simulink model "ScaraRobotApresentacao2023"  (R2024a)
settings: Solver=VariableStepAuto  StartTime=0.0  StopTime=200  RelTol=1e-3
model workspace: external: MATLAB File C:\Users\lucas\OneDrive\Documents\MATLAB\Robotica_2023b\ScaraRobot_DataFile.m (data not in the file)
values from neighbouring files (symbols this model uses):
  I = cell(1,n)    [calcularDinamica.m]    (also in inicializacaoAntropomorfico.m = {I1, I2, I3, I4, I5, I6, I7})
  L = [L1, L2, L3, L4, L5, L6, L7]    [inicializacaoAntropomorfico.m]
  Lcm = {Lcm1, Lcm2, Lcm3, Lcm4, Lcm5, Lcm6, Lcm7}    [inicializacaoAntropomorfico.m]
  m = [m1, m2, m3, m4, m5, m6, m7]    [inicializacaoAntropomorfico.m]
  Pf = [  0.05    [inicializacaoAntropomorfico.m]
  Pi = [  0.2    [inicializacaoAntropomorfico.m]
  Raio = [0]    [inicializacaoAntropomorfico.m]
  Sentido = [0]    [inicializacaoAntropomorfico.m]
  Tipo = [1]    [inicializacaoAntropomorfico.m]
undefined symbols (not defined in the file or in its folder): Lx1, Lx2, smiData, X, Y, Z
libraries: sm_lib x25, nesl_utility x5
(part 2 of 10)

== matlab function ScaraRobotApresentacao2023/Dinamica/MATLAB Function ==
  data: M output; I parameter; L parameter; Lcm parameter; Q input
function M = func_M(I, L, Lcm, Q)
%func_M
%    OUT1 = func_M(Ixx2,Ixx3,Ixx4,Ixx5,Ixx6,Ixy2,Ixy3,Ixy4,Ixy5,Ixy6,Ixz2,Ixz3,Ixz4,Ixz5,Ixz6,Iyx2,Iyx3,Iyx4,Iyx5,Iyx6,Iyy2,Iyy3,Iyy4,Iyy5,Iyy6,Iyz2,Iyz3,Iyz4,Iyz5,Iyz6,Izx2,Izx3,Izx4,Izx5,Izx6,Izy2,Izy3,Izy4,Izy5,Izy6,Izz1,Izz2,Izz3,Izz4,Izz5,Izz6,Lx2,Lx3,Lxcm1,Lxcm2,Lxcm3,Lxcm4,Lxcm5,Lxcm6,Lycm1,Lycm2,Lycm3,Lycm4,Lycm5,Lycm6,Lz4,Lz5,Lzcm2,Lzcm3,Lzcm4,Lzcm5,Lzcm6,Q1,Q2,Q3,Q4,Q5,Q6,M1,M2,M3,M4,M5,M6)
    
%    This function was generated by the Symbolic Math Toolbox version 24.1.
%    30-Apr-2025 07:30:44

Q1  = Q(1);
Q2  = Q(2);
Q3  = Q(3);
Q4  = Q(4);
Q5  = Q(5);
Q6  = Q(6);

Lx1 = L{1}(1);
Ly1 = L{1}(2);
Lz1 = L{1}(3);

Lx2 = L{2}(1);
Ly2 = L{2}(2);
Lz2 = L{2}(3);

Lx3 = L{3}(1);
Ly3 = L{3}(2);
Lz3 = L{3}(3);

Lx4 = L{4}(1);
Ly4 = L{4}(2);
Lz4 = L{4}(3);

Lx5 = L{5}(1);
Ly5 = L{5}(2);
Lz5 = L{5}(3);

Lx6 = L{6}(1);
Ly6 = L{6}(2);
Lz6 = L{6}(3);

Lxcm1 = Lcm{1}(1);
Lycm1 = Lcm{1}(2);
Lzcm1 = Lcm{1}(3);

Lxcm2 = Lcm{2}(1);
Lycm2 = Lcm{2}(2);
Lzcm2 = Lcm{2}(3);

Lxcm3 = Lcm{3}(1);
Lycm3 = Lcm{3}(2);
Lzcm3 = Lcm{3}(3);

Lxcm4 = Lcm{4}(1);
Lycm4 = Lcm{4}(2);
Lzcm4 = Lcm{4}(3);

Lxcm5 = Lcm{5}(1);
Lycm5 = Lcm{5}(2);
Lzcm5 = Lcm{5}(3);

Lxcm6 = Lcm{6}(1);
Lycm6 = Lcm{6}(2);
Lzcm6 = Lcm{6}(3);

Ixx1 = I{1}(1,1);
Ixy1 = I{1}(1,2);
Ixz1 = I{1}(1,3);
Iyx1 = I{1}(2,1);
Iyy1 = I{1}(2,2);
Iyz1 = I{1}(2,3);
Izx1 = I{1}(3,1);
Izy1 = I{1}(3,2);
Izz1 = I{1}(3,3);

Ixx2 = I{2}(1,1);
Ixy2 = I{2}(1,2);
Ixz2 = I{2}(1,3);
Iyx2 = I{2}(2,1);
Iyy2 = I{2}(2,2);
Iyz2 = I{2}(2,3);
Izx2 = I{2}(3,1);
Izy2 = I{2}(3,2);
Izz2 = I{2}(3,3);

Ixx3 = I{3}(1,1);
Ixy3 = I{3}(1,2);
Ixz3 = I{3}(1,3);
Iyx3 = I{3}(2,1);
Iyy3 = I{3}(2,2);
Iyz3 = I{3}(2,3);
Izx3 = I{3}(3,1);
Izy3 = I{3}(3,2);
Izz3 = I{3}(3,3);

Ixx4 = I{4}(1,1);
Ixy4 = I{4}(1,2);
Ixz4 = I{4}(1,3);
Iyx4 = I{4}(2,1);
Iyy4 = I{4}(2,2);
Iyz4 = I{4}(2,3);
Izx4 = I{4}(3,1);
Izy4 = I{4}(3,2);
Izz4 = I{4}(3,3);

Ixx5 = I{5}(1,1);
Ixy5 = I{5}(1,2);
Ixz5 = I{5}(1,3);
Iyx5 = I{5}(2,1);
Iyy5 = I{5}(2,2);
Iyz5 = I{5}(2,3);
Izx5 = I{5}(3,1);
Izy5 = I{5}(3,2);
Izz5 = I{5}(3,3);

Ixx6 = I{6}(1,1);
Ixy6 = I{6}(1,2);
Ixz6 = I{6}(1,3);
Iyx6 = I{6}(2,1);
Iyy6 = I{6}(2,2);
Iyz6 = I{6}(2,3);
Izx6 = I{6}(3,1);
Izy6 = I{6}(3,2);
Izz6 = I{6}(3,3);


t2 = cos(Q1);
t3 = cos(Q2);
t4 = cos(Q3);
t5 = cos(Q4);
t6 = cos(Q5);
t7 = cos(Q6);
t8 = sin(Q1);
t9 = sin(Q2);
t10 = sin(Q3);
t11 = sin(Q4);
t12 = sin(Q5);
t13 = sin(Q6);
t14 = Q2+Q3;
t15 = Lx2.^2;
t16 = Lx3.^2;
t17 = Lxcm3.^2;
t18 = Lxcm4.^2;
t19 = Lxcm5.^2;
t20 = Lxcm6.^2;
t21 = Lycm4.^2;
t22 = Lycm5.^2;
t23 = Lycm6.^2;
t24 = Lz4.^2;
t25 = Lz5.^2;
t26 = Lzcm3.^2;
t27 = Lzcm4.^2;
t28 = Lzcm5.^2;
t29 = Lzcm6.^2;
t30 = Q4.*2.0;
t31 = Q5.*2.0;
t32 = Q6.*2.0;
t45 = Lz5.*Lzcm6.*m6.*2.0;
t33 = cos(t32);
t34 = t5.^2;
t35 = t6.^2;
t36 = t7.^2;
t37 = sin(t30);
t38 = sin(t31);
t39 = sin(t32);
t40 = Ixx6.*t5;
t41 = Iyy5.*t5;
t42 = Izz6.*t6;
t43 = cos(t14);
t44 = sin(t14);
t46 = m4.*t16;
t47 = m5.*t16;
t48 = m6.*t16;
t49 = m3.*t17;
t50 = m5.*t19;
t51 = m6.*t20;
t52 = m4.*t21;
t53 = m5.*t22;
t54 = m6.*t23;
t55 = m5.*t24;
t56 = m6.*t24;
t57 = m6.*t25;
t58 = m3.*t26;
t59 = m4.*t27;
t60 = m5.*t28;
t61 = m6.*t29;
t62 = t2.*t5;
t63 = t2.*t11;
t64 = t5.*t8;
t65 = t8.*t11;
t66 = Ixx5.*t3.*t4;
t67 = Iyy6.*t3.*t4;
t68 = Izz4.*t3.*t4;
t69 = Lx2.*t2.*t3;
t70 = Lx2.*Lx3.*m4.*t4;
t71 = Lx2.*Lx3.*m5.*t4;
t72 = Lx2.*Lx3.*m6.*t4;
t73 = Lx2.*Lxcm3.*m3.*t4;
t74 = Lx3.*Lxcm5.*m5.*t6;
t75 = Lycm5.*Lz4.*m5.*t5;
t76 = Lycm6.*Lz5.*m6.*t7;
t77 = Lycm2.*Lzcm2.*m2.*t3;
t78 = Lycm4.*Lzcm4.*m4.*t5;
t79 = Lycm5.*Lzcm5.*m5.*t6;
t80 = Lycm6.*Lzcm6.*m6.*t7;
t81 = Lx2.*t3.*t8;
t82 = Lx2.*Lycm3.*m3.*t9;
t83 = Lxcm2.*Lycm2.*m2.*t9;
t84 = Lxcm5.*Lycm5.*m5.*t12;
t85 = Lxcm6.*Lycm6.*m6.*t12;
t86 = Lx2.*Lz4.*m5.*t10;
t87 = Lx2.*Lz4.*m6.*t10;
t88 = Lx3.*Lz5.*m6.*t12;
t89 = Lx2.*Lzcm3.*m3.*t10;
t90 = Lx2.*Lzcm4.*m4.*t10;
t91 = Lx3.*Lzcm5.*m5.*t12;
t92 = Lx3.*Lzcm6.*m6.*t12;
t93 = Lxcm6.*Lz5.*m6.*t13;
t94 = Lxcm4.*Lzcm4.*m4.*t11;
t95 = Lxcm5.*Lzcm5.*m5.*t11;
t96 = Lxcm6.*Lzcm6.*m6.*t13;
t97 = Ixx5.*t9.*t10;
t98 = Iyy6.*t9.*t10;
t99 = Izz4.*t9.*t10;
t100 = Izz6.*t11.*t12;
t111 = Lx3.*Lxcm4.*m4.*t5.*2.0;
t112 = Lz4.*Lz5.*m6.*t6.*2.0;
t113 = Lz4.*Lzcm5.*m5.*t6.*2.0;
t114 = Lz4.*Lzcm6.*m6.*t6.*2.0;
t115 = t5.*t45;
t116 = Lx3.*Lycm4.*m4.*t11.*2.0;
t117 = Lx3.*Lycm5.*m5.*t11.*2.0;
t118 = Lxcm5.*Lz4.*m5.*t12.*2.0;
t126 = (Iyz2.*t3)./2.0;
t127 = (Iyz4.*t5)./2.0;
t128 = (Iyz5.*t6)./2.0;
t129 = (Iyz6.*t7)./2.0;
t130 = (Izy2.*t3)./2.0;
t131 = (Izy4.*t5)./2.0;
t132 = (Izy5.*t6)./2.0;
t133 = (Izy6.*t7)./2.0;
t134 = (Ixy2.*t9)./2.0;
t135 = (Ixy5.*t12)./2.0;
t136 = (Ixy6.*t12)./2.0;
t137 = (Ixz4.*t11)./2.0;
t138 = (Ixz5.*t11)./2.0;
t139 = (Ixz6.*t13)./2.0;
t140 = (Iyx2.*t9)./2.0;
t141 = (Iyx5.*t12)./2.0;
t142 = (Iyx6.*t12)./2.0;
t143 = (Izx4.*t11)./2.0;
t144 = (Izx5.*t11)./2.0;
t145 = (Izx6.*t13)./2.0;
t147 = t2.*t3.*t4;
t149 = t2.*t3.*t10;
t150 = t2.*t4.*t9;
t151 = t3.*t4.*t8;
t152 = t2.*t9.*t10;
t153 = t3.*t8.*t10;
t154 = t4.*t8.*t9;
t155 = t8.*t9.*t10;
t203 = Lx2.*Lxcm4.*m4.*t3.*t5;
t204 = Lx2.*Lxcm4.*m4.*t4.*t5;
t205 = Lx2.*Lxcm5.*m5.*t4.*t6;
t206 = Lx3.*Lxcm6.*m6.*t6.*t7;
t207 = Lycm6.*Lz4.*m6.*t5.*t7;
t210 = Lycm3.*Lzcm3.*m3.*t3.*t4;
t214 = Lz4.*Lz5.*m6.*t5.*t6;
t215 = Lz4.*Lzcm5.*m5.*t5.*t6;
t216 = Lz4.*Lzcm6.*m6.*t5.*t6;
t217 = Ixy5.*t5.*t6.*t11;
t218 = Ixy6.*t5.*t6.*t11;
t219 = Ixy6.*t5.*t7.*t13;
t220 = Ixz6.*t6.*t7.*t12;
t221 = Iyx5.*t5.*t6.*t11;
t222 = Iyx6.*t5.*t6.*t11;
t223 = Iyx6.*t5.*t7.*t13;
t224 = Izx6.*t6.*t7.*t12;
t225 = Lx2.*Lycm4.*m4.*t3.*t11;
t226 = Lx2.*Lycm4.*m4.*t5.*t9;
t227 = Lx2.*Lycm4.*m4.*t4.*t11;
t228 = Lx2.*Lycm4.*m4.*t5.*t10;
t229 = Lx2.*Lycm5.*m5.*t3.*t11;
t230 = Lx2.*Lycm5.*m5.*t5.*t9;
t231 = Lx2.*Lycm5.*m5.*t4.*t11;
t232 = Lx2.*Lycm5.*m5.*t5.*t10;
t233 = Lx3.*Lycm6.*m6.*t6.*t13;
t234 = Lx3.*Lycm6.*m6.*t7.*t12;
t235 = Lxcm3.*Lycm3.*m3.*t3.*t10;
t236 = Lxcm3.*Lycm3.*m3.*t4.*t9;
t237 = Lxcm4.*Lycm4.*m4.*t3.*t10;
t238 = Lxcm4.*Lycm4.*m4.*t4.*t9;
t240 = Lxcm5.*Lycm5.*m5.*t6.*t11;
t242 = Lxcm6.*Lycm6.*m6.*t6.*t11;
t243 = Lx2.*Lz5.*m6.*t4.*t12;
t244 = Lx2.*Lz5.*m6.*t6.*t10;
t245 = Lx2.*Lzcm5.*m5.*t4.*t12;
t246 = Lx2.*Lzcm5.*m5.*t6.*t10;
t247 = Lx2.*Lzcm6.*m6.*t4.*t12;
t248 = Lx2.*Lzcm6.*m6.*t6.*t10;
t249 = Lxcm5.*Lz4.*m5.*t5.*t12;
t250 = Lxcm5.*Lz4.*m5.*t6.*t11;
t251 = Lxcm6.*Lz4.*m6.*t5.*t13;
t252 = Lxcm6.*Lz4.*m6.*t7.*t11;
t254 = Lxcm6.*Lz5.*m6.*t7.*t11;
t256 = Lxcm6.*Lz5.*m6.*t7.*t12;
t258 = Lxcm6.*Lzcm6.*m6.*t7.*t11;
t260 = Lxcm6.*Lzcm6.*m6.*t7.*t12;
t261 = Ixx6.*t3.*t10.*t11;
t262 = Ixx6.*t4.*t9.*t11;
t263 = Ixx5.*t6.*t11.*t12;
t264 = Ixx6.*t7.*t12.*t13;
t265 = Iyy5.*t3.*t10.*t11;
t266 = Iyy5.*t4.*t9.*t11;
t267 = Iyy6.*t6.*t11.*t12;
t268 = Iyy6.*t7.*t12.*t13;
t269 = Iyz5.*t5.*t11.*t12;
t270 = Iyz6.*t6.*t12.*t13;
t271 = Izy5.*t5.*t11.*t12;
t272 = Izy6.*t6.*t12.*t13;
t274 = Izz5.*t6.*t11.*t12;
t276 = Lx2.*Lxcm4.*m4.*t9.*t11;
t277 = Lx2.*Lxcm4.*m4.*t10.*t11;
t278 = Lx2.*Lxcm5.*m5.*t10.*t12;
t279 = Lx3.*Lxcm6.*m6.*t12.*t13;
t280 = Lycm6.*Lz4.*m6.*t11.*t13;
t281 = Lycm6.*Lz5.*m6.*t11.*t13;
t282 = Lycm6.*Lz5.*m6.*t12.*t13;
t283 = Lycm3.*Lzcm3.*m3.*t9.*t10;
t284 = Lycm5.*Lzcm5.*m5.*t11.*t12;
t285 = Lycm6.*Lzcm6.*m6.*t11.*t13;
t286 = Lycm6.*Lzcm6.*m6.*t12.*t13;
t287 = Lz4.*Lz5.*m6.*t11.*t12;
t288 = Lz4.*Lzcm5.*m5.*t11.*t12;
t289 = Lz4.*Lzcm6.*m6.*t11.*t12;
t290 = m4.*t9.*t10.*t18;
t299 = (Iyz3.*t3.*t4)./2.0;
t303 = (Izy3.*t3.*t4)./2.0;
t307 = (Ixy3.*t3.*t10)./2.0;
t308 = (Ixy3.*t4.*t9)./2.0;
t309 = (Ixy4.*t3.*t10)./2.0;
t310 = (Ixy4.*t4.*t9)./2.0;
t312 = (Ixy5.*t6.*t11)./2.0;
t314 = (Ixy6.*t6.*t11)./2.0;
t316 = (Ixz6.*t7.*t11)./2.0;
t318 = (Ixz6.*t7.*t12)./2.0;
t319 = (Iyx3.*t3.*t10)./2.0;
t320 = (Iyx3.*t4.*t9)./2.0;
t321 = (Iyx4.*t3.*t10)./2.0;
t322 = (Iyx4.*t4.*t9)./2.0;
t324 = (Iyx5.*t6.*t11)./2.0;
t326 = (Iyx6.*t6.*t11)./2.0;
t328 = (Izx6.*t7.*t11)./2.0;
t330 = (Izx6.*t7.*t12)./2.0;
t331 = (Iyz3.*t9.*t10)./2.0;
t332 = (Iyz5.*t11.*t12)./2.0;
t333 = (Iyz6.*t11.*t13)./2.0;
t334 = (Iyz6.*t12.*t13)./2.0;
t335 = (Izy3.*t9.*t10)./2.0;
t336 = (Izy5.*t11.*t12)./2.0;
t337 = (Izy6.*t11.*t13)./2.0;
t338 = (Izy6.*t12.*t13)./2.0;
t366 = t3.*t4.*t45;
t367 = Lx3.*Lycm6.*m6.*t7.*t11.*2.0;
t371 = Lxcm6.*Lz4.*m6.*t7.*t12.*2.0;
t372 = m4.*t3.*t4.*t18;
t379 = Lx3.*Lxcm6.*m6.*t11.*t13.*2.0;
t380 = Lycm6.*Lz4.*m6.*t12.*t13.*2.0;
t381 = t9.*t10.*t45;
t383 = Iyz5.*t5.*t6.*(-1.0./2.0);
t384 = Iyz6.*t5.*t7.*(-1.0./2.0);
t385 = Iyz6.*t6.*t7.*(-1.0./2.0);
t387 = Izy5.*t5.*t6.*(-1.0./2.0);
t388 = Izy6.*t5.*t7.*(-1.0./2.0);
t389 = Izy6.*t6.*t7.*(-1.0./2.0);
t393 = Ixy6.*t5.*t12.*(-1.0./2.0);
t394 = Ixz6.*t5.*t13.*(-1.0./2.0);
t395 = Ixz6.*t6.*t13.*(-1.0./2.0);
t399 = Iyx6.*t5.*t12.*(-1.0./2.0);
t400 = Izx6.*t5.*t13.*(-1.0./2.0);
t401 = Izx6.*t6.*t13.*(-1.0./2.0);
t441 = Lx3.*Lxcm4.*m4.*t3.*t4.*t5;
t442 = Lx2.*Lxcm5.*m5.*t3.*t5.*t6;
t444 = Lx2.*Lxcm6.*m6.*t3.*t5.*t7;
t445 = Lx2.*Lxcm6.*m6.*t4.*t6.*t7;
t454 = Ixy6.*t3.*t4.*t7.*t13;
t455 = Ixz5.*t3.*t4.*t6.*t12;
t456 = Iyx6.*t3.*t4.*t7.*t13;
t457 = Izx5.*t3.*t4.*t6.*t12;
t458 = Lx3.*Lycm4.*m4.*t3.*t4.*t11;
t459 = Lx3.*Lycm4.*m4.*t3.*t5.*t10;
t460 = Lx3.*Lycm4.*m4.*t4.*t5.*t9;
t461 = Lx3.*Lycm5.*m5.*t3.*t4.*t11;
t462 = Lx3.*Lycm5.*m5.*t3.*t5.*t10;
t463 = Lx3.*Lycm5.*m5.*t4.*t5.*t9;
t464 = Lx2.*Lycm6.*m6.*t3.*t5.*t13;
t465 = Lx2.*Lycm6.*m6.*t3.*t7.*t11;
t466 = Lx2.*Lycm6.*m6.*t5.*t7.*t9;
t467 = Lx2.*Lycm6.*m6.*t4.*t7.*t11;
t468 = Lx2.*Lycm6.*m6.*t5.*t7.*t10;
t469 = Lx2.*Lycm6.*m6.*t4.*t6.*t13;
t470 = Lx2.*Lycm6.*m6.*t4.*t7.*t12;
t472 = Lxcm5.*Lycm5.*m5.*t3.*t6.*t10;
t473 = Lxcm5.*Lycm5.*m5.*t4.*t6.*t9;
t475 = Lxcm6.*Lycm6.*m6.*t3.*t6.*t10;
t476 = Lxcm6.*Lycm6.*m6.*t4.*t6.*t9;
t477 = Lx2.*Lz5.*m6.*t3.*t5.*t12;
t478 = Lx2.*Lz5.*m6.*t3.*t6.*t11;
t481 = Lx2.*Lzcm5.*m5.*t3.*t5.*t12;
t482 = Lx2.*Lzcm5.*m5.*t3.*t6.*t11;
t485 = Lx2.*Lzcm6.*m6.*t3.*t5.*t12;
t486 = Lx2.*Lzcm6.*m6.*t3.*t6.*t11;
t490 = Lxcm6.*Lz4.*m6.*t5.*t7.*t12;
t495 = Lxcm4.*Lzcm4.*m4.*t3.*t5.*t10;
t496 = Lxcm4.*Lzcm4.*m4.*t4.*t5.*t9;
t498 = Lxcm5.*Lzcm5.*m5.*t3.*t5.*t10;
t499 = Lxcm5.*Lzcm5.*m5.*t4.*t5.*t9;
t502 = Ixx4.*t3.*t5.*t10.*t11;
t503 = Ixx4.*t4.*t5.*t9.*t11;
t507 = Ixx6.*t6.*t7.*t11.*t13;
t508 = Iyy4.*t3.*t5.*t10.*t11;
t509 = Iyy4.*t4.*t5.*t9.*t11;
t513 = Iyy6.*t6.*t7.*t11.*t13;
t514 = Iyz6.*t5.*t7.*t11.*t12;
t515 = Izy6.*t5.*t7.*t11.*t12;
t516 = Izz5.*t3.*t5.*t10.*t11;
t517 = Izz5.*t4.*t5.*t9.*t11;
t518 = Izz6.*t3.*t5.*t10.*t11;
t519 = Izz6.*t4.*t5.*t9.*t11;
t520 = Izz6.*t3.*t5.*t10.*t12;
t521 = Izz6.*t4.*t5.*t9.*t12;
t522 = Lx3.*Lxcm4.*m4.*t3.*t10.*t11;
t523 = Lx3.*Lxcm4.*m4.*t4.*t9.*t11;
t524 = Lx3.*Lxcm4.*m4.*t5.*t9.*t10;
t525 = Lx2.*Lxcm5.*m5.*t3.*t11.*t12;
t526 = Lx2.*Lxcm5.*m5.*t6.*t9.*t11;
t528 = Lx2.*Lxcm5.*m5.*t6.*t10.*t11;
t529 = Lx2.*Lxcm6.*m6.*t3.*t11.*t13;
t530 = Lx2.*Lxcm6.*m6.*t5.*t9.*t13;
t531 = Lx2.*Lxcm6.*m6.*t4.*t11.*t13;
t532 = Lx2.*Lxcm6.*m6.*t5.*t10.*t13;
t533 = Lx2.*Lxcm6.*m6.*t7.*t10.*t11;
t534 = Lx2.*Lxcm6.*m6.*t4.*t12.*t13;
t535 = Lx2.*Lxcm6.*m6.*t7.*t10.*t12;
t536 = Lycm5.*Lz4.*m5.*t3.*t10.*t11;
t537 = Lycm5.*Lz4.*m5.*t4.*t9.*t11;
t539 = Lycm6.*Lz4.*m6.*t5.*t12.*t13;
t543 = Lycm4.*Lzcm4.*m4.*t3.*t10.*t11;
t544 = Lycm4.*Lzcm4.*m4.*t4.*t9.*t11;
t546 = Lycm5.*Lzcm5.*m5.*t3.*t10.*t12;
t547 = Lycm5.*Lzcm5.*m5.*t4.*t9.*t12;
t551 = Ixy6.*t7.*t9.*t10.*t13;
t552 = Ixz5.*t6.*t9.*t10.*t12;
t553 = Ixz6.*t5.*t11.*t12.*t13;
t554 = Iyx6.*t7.*t9.*t10.*t13;
t555 = Izx5.*t6.*t9.*t10.*t12;
t556 = Izx6.*t5.*t11.*t12.*t13;
t557 = Lx3.*Lycm4.*m4.*t9.*t10.*t11;
t558 = Lx3.*Lycm5.*m5.*t9.*t10.*t11;
t559 = Lx2.*Lycm6.*m6.*t10.*t11.*t13;
t560 = Lx2.*Lycm6.*m6.*t10.*t12.*t13;
t563 = Lx2.*Lz5.*m6.*t9.*t11.*t12;
t564 = Lx2.*Lz5.*m6.*t10.*t11.*t12;
t565 = Lx2.*Lzcm5.*m5.*t9.*t11.*t12;
t566 = Lx2.*Lzcm5.*m5.*t10.*t11.*t12;
t567 = Lx2.*Lzcm6.*m6.*t9.*t11.*t12;
t568 = Lx2.*Lzcm6.*m6.*t10.*t11.*t12;
t637 = Lz5.*Lzcm6.*m6.*t9.*t10.*-2.0;
t661 = Lxcm6.*Lycm6.*m6.*t5.*t7.*t13.*2.0;
t669 = t3.*t10.*t11.*t45;
t670 = t4.*t9.*t11.*t45;
t698 = (Ixy5.*t3.*t6.*t10)./2.0;
t699 = (Ixy5.*t4.*t6.*t9)./2.0;
t701 = (Ixy6.*t3.*t6.*t10)./2.0;
t702 = (Ixy6.*t4.*t6.*t9)./2.0;
t704 = (Ixz4.*t3.*t5.*t10)./2.0;
t705 = (Ixz4.*t4.*t5.*t9)./2.0;
t707 = (Ixz5.*t3.*t5.*t10)./2.0;
t708 = (Ixz5.*t4.*t5.*t9)./2.0;
t712 = (Iyx5.*t3.*t6.*t10)./2.0;
t713 = (Iyx5.*t4.*t6.*t9)./2.0;
t715 = (Iyx6.*t3.*t6.*t10)./2.0;
t716 = (Iyx6.*t4.*t6.*t9)./2.0;
t718 = (Izx4.*t3.*t5.*t10)./2.0;
t719 = (Izx4.*t4.*t5.*t9)./2.0;
t721 = (Izx5.*t3.*t5.*t10)./2.0;
t722 = (Izx5.*t4.*t5.*t9)./2.0;
t725 = (Iyz4.*t3.*t10.*t11)./2.0;
t726 = (Iyz4.*t4.*t9.*t11)./2.0;
t728 = (Iyz5.*t3.*t10.*t12)./2.0;
t729 = (Iyz5.*t4.*t9.*t12)./2.0;
t733 = (Izy4.*t3.*t10.*t11)./2.0;
t734 = (Izy4.*t4.*t9.*t11)./2.0;
t736 = (Izy5.*t3.*t10.*t12)./2.0;
t737 = (Izy5.*t4.*t9.*t12)./2.0;
t765 = Lx3.*Lxcm6.*m6.*t3.*t4.*t5.*t7;
t778 = Lx3.*Lycm6.*m6.*t3.*t4.*t5.*t13;
t779 = Lx3.*Lycm6.*m6.*t3.*t4.*t7.*t11;
t780 = Lx3.*Lycm6.*m6.*t3.*t5.*t7.*t10;
t781 = Lx3.*Lycm6.*m6.*t4.*t5.*t7.*t9;
t793 = Lx3.*Lz5.*m6.*t3.*t4.*t6.*t11;
t795 = Lx3.*Lzcm5.*m5.*t3.*t4.*t6.*t11;
t797 = Lxcm5.*Lz4.*m5.*t3.*t5.*t6.*t10;
t798 = Lxcm5.*Lz4.*m5.*t4.*t5.*t6.*t9;
t800 = Lx3.*Lzcm6.*m6.*t3.*t4.*t6.*t11;
t802 = Lxcm6.*Lz4.*m6.*t3.*t5.*t7.*t10;
t803 = Lxcm6.*Lz4.*m6.*t4.*t5.*t7.*t9;
t805 = Lxcm6.*Lz5.*m6.*t3.*t5.*t7.*t10;
t806 = Lxcm6.*Lz5.*m6.*t4.*t5.*t7.*t9;
t810 = Lxcm6.*Lzcm6.*m6.*t3.*t5.*t7.*t10;
t811 = Lxcm6.*Lzcm6.*m6.*t4.*t5.*t7.*t9;
t815 = Ixx5.*t3.*t5.*t6.*t10.*t12;
t816 = Ixx5.*t4.*t5.*t6.*t9.*t12;
t818 = Ixx6.*t3.*t6.*t7.*t10.*t13;
t819 = Ixx6.*t4.*t6.*t7.*t9.*t13;
t821 = Iyy6.*t3.*t5.*t6.*t10.*t12;
t822 = Iyy6.*t4.*t5.*t6.*t9.*t12;
t824 = Iyy6.*t3.*t6.*t7.*t10.*t13;
t825 = Iyy6.*t4.*t6.*t7.*t9.*t13;
t829 = Izz5.*t3.*t5.*t6.*t10.*t12;
t830 = Izz5.*t4.*t5.*t6.*t9.*t12;
t834 = Lx3.*Lxcm5.*m5.*t3.*t4.*t11.*t12;
t838 = Lx3.*Lxcm6.*m6.*t3.*t4.*t11.*t13;
t839 = Lx3.*Lxcm6.*m6.*t3.*t5.*t10.*t13;
t840 = Lx3.*Lxcm6.*m6.*t4.*t5.*t9.*t13;
t841 = Lx3.*Lxcm6.*m6.*t5.*t7.*t9.*t10;
t843 = Lx2.*Lxcm6.*m6.*t3.*t7.*t11.*t12;
t844 = Lx2.*Lxcm6.*m6.*t6.*t7.*t9.*t11;
t848 = Lycm6.*Lz4.*m6.*t3.*t5.*t10.*t13;
t849 = Lycm6.*Lz4.*m6.*t3.*t7.*t10.*t11;
t850 = Lycm6.*Lz4.*m6.*t4.*t5.*t9.*t13;
t851 = Lycm6.*Lz4.*m6.*t4.*t7.*t9.*t11;
t854 = Lycm6.*Lz5.*m6.*t3.*t5.*t10.*t13;
t856 = Lycm6.*Lz5.*m6.*t4.*t5.*t9.*t13;
t868 = Lycm6.*Lzcm6.*m6.*t3.*t5.*t10.*t13;
t870 = Lycm6.*Lzcm6.*m6.*t4.*t5.*t9.*t13;
t877 = Lz4.*Lz5.*m6.*t3.*t5.*t10.*t12;
t878 = Lz4.*Lz5.*m6.*t3.*t6.*t10.*t11;
t879 = Lz4.*Lz5.*m6.*t4.*t5.*t9.*t12;
t880 = Lz4.*Lz5.*m6.*t4.*t6.*t9.*t11;
t882 = Lz4.*Lzcm5.*m5.*t3.*t5.*t10.*t12;
t883 = Lz4.*Lzcm5.*m5.*t3.*t6.*t10.*t11;
t884 = Lz4.*Lzcm5.*m5.*t4.*t5.*t9.*t12;
t885 = Lz4.*Lzcm5.*m5.*t4.*t6.*t9.*t11;
t887 = Lz4.*Lzcm6.*m6.*t3.*t5.*t10.*t12;
t888 = Lz4.*Lzcm6.*m6.*t3.*t6.*t10.*t11;
t889 = Lz4.*Lzcm6.*m6.*t4.*t5.*t9.*t12;
t890 = Lz4.*Lzcm6.*m6.*t4.*t6.*t9.*t11;
t891 = Ixy6.*t3.*t7.*t10.*t11.*t13;
t892 = Ixy6.*t4.*t7.*t9.*t11.*t13;
t893 = Ixy6.*t6.*t7.*t11.*t12.*t13;
t895 = Iyx6.*t3.*t7.*t10.*t11.*t13;
t896 = Iyx6.*t4.*t7.*t9.*t11.*t13;
t897 = Iyx6.*t6.*t7.*t11.*t12.*t13;
t899 = Lx3.*Lycm6.*m6.*t5.*t9.*t10.*t13;
t900 = Lx3.*Lycm6.*m6.*t7.*t9.*t10.*t11;
t901 = Lx2.*Lycm6.*m6.*t3.*t11.*t12.*t13;
t902 = Lx2.*Lycm6.*m6.*t6.*t9.*t11.*t13;
t914 = Lx3.*Lz5.*m6.*t6.*t9.*t10.*t11;
t918 = Lx3.*Lzcm5.*m5.*t6.*t9.*t10.*t11;
t919 = Lxcm5.*Lz4.*m5.*t3.*t10.*t11.*t12;
t920 = Lxcm5.*Lz4.*m5.*t4.*t9.*t11.*t12;
t925 = Lx3.*Lzcm6.*m6.*t6.*t9.*t10.*t11;
t926 = Lxcm6.*Lz4.*m6.*t3.*t10.*t11.*t13;
t927 = Lxcm6.*Lz4.*m6.*t4.*t9.*t11.*t13;
t951 = Lx3.*Lxcm5.*m5.*t9.*t10.*t11.*t12;
t952 = Lx3.*Lxcm6.*m6.*t9.*t10.*t11.*t13;
t1023 = Lz5.*Lzcm6.*m6.*t6.*t11.*t12.*-2.0;
t1037 = Iyz4.*t3.*t4.*t5.*(-1.0./2.0);
t1038 = Iyz5.*t3.*t4.*t6.*(-1.0./2.0);
t1040 = Izy4.*t3.*t4.*t5.*(-1.0./2.0);
t1041 = Izy5.*t3.*t4.*t6.*(-1.0./2.0);
t1049 = Ixy6.*t3.*t4.*t12.*(-1.0./2.0);
t1050 = Ixz4.*t3.*t4.*t11.*(-1.0./2.0);
t1054 = Ixz6.*t6.*t7.*t11.*(-1.0./2.0);
t1057 = Iyx6.*t3.*t4.*t12.*(-1.0./2.0);
t1058 = Izx4.*t3.*t4.*t11.*(-1.0./2.0);
t1062 = Izx6.*t6.*t7.*t11.*(-1.0./2.0);
t1067 = Iyz6.*t7.*t11.*t12.*(-1.0./2.0);
t1072 = Izy6.*t7.*t11.*t12.*(-1.0./2.0);
t1095 = Ixy5.*t9.*t10.*t12.*(-1.0./2.0);
t1096 = Ixz5.*t9.*t10.*t11.*(-1.0./2.0);
t1097 = Ixz6.*t11.*t12.*t13.*(-1.0./2.0);
t1098 = Iyx5.*t9.*t10.*t12.*(-1.0./2.0);
t1099 = Izx5.*t9.*t10.*t11.*(-1.0./2.0);
t1100 = Izx6.*t11.*t12.*t13.*(-1.0./2.0);
t1124 = Lxcm6.*Lycm6.*m6.*t3.*t4.*t7.*t13.*2.0;
t1125 = Lxcm5.*Lzcm5.*m5.*t3.*t4.*t6.*t12.*2.0;
t1132 = Lxcm6.*Lycm6.*m6.*t7.*t9.*t10.*t13.*2.0;
t1134 = Lxcm5.*Lzcm5.*m5.*t6.*t9.*t10.*t12.*2.0;
t1136 = m4.*t3.*t5.*t10.*t11.*t18;
t1137 = m4.*t4.*t5.*t9.*t11.*t18;
t1169 = (Ixz6.*t3.*t5.*t7.*t10)./2.0;
t1170 = (Ixz6.*t4.*t5.*t7.*t9)./2.0;
t1180 = (Izx6.*t3.*t5.*t7.*t10)./2.0;
t1181 = (Izx6.*t4.*t5.*t7.*t9)./2.0;
t1191 = (Iyz6.*t3.*t5.*t10.*t13)./2.0;
t1193 = (Iyz6.*t4.*t5.*t9.*t13)./2.0;
t1205 = (Izy6.*t3.*t5.*t10.*t13)./2.0;
t1207 = (Izy6.*t4.*t5.*t9.*t13)./2.0;
t1286 = Lx3.*Lxcm6.*m6.*t3.*t4.*t7.*t11.*t12;
t1311 = Ixz5.*t3.*t5.*t6.*t10.*t11.*t12;
t1312 = Ixz5.*t4.*t5.*t6.*t9.*t11.*t12;
t1315 = Izx5.*t3.*t5.*t6.*t10.*t11.*t12;
t1316 = Izx5.*t4.*t5.*t6.*t9.*t11.*t12;
t1317 = Lx3.*Lycm6.*m6.*t3.*t4.*t11.*t12.*t13;
t1344 = Lx3.*Lxcm6.*m6.*t7.*t9.*t10.*t11.*t12;
t1354 = Lx3.*Lycm6.*m6.*t9.*t10.*t11.*t12.*t13;
t1466 = Ixy6.*t3.*t5.*t6.*t10.*(-1.0./2.0);
t1467 = Ixy6.*t4.*t5.*t6.*t9.*(-1.0./2.0);
t1472 = Iyx6.*t3.*t5.*t6.*t10.*(-1.0./2.0);
t1473 = Iyx6.*t4.*t5.*t6.*t9.*(-1.0./2.0);
t1478 = Iyz5.*t3.*t6.*t10.*t11.*(-1.0./2.0);
t1479 = Iyz5.*t4.*t6.*t9.*t11.*(-1.0./2.0);
t1480 = Iyz6.*t3.*t4.*t11.*t13.*(-1.0./2.0);
t1481 = Iyz6.*t3.*t7.*t10.*t11.*(-1.0./2.0);
t1482 = Iyz6.*t4.*t7.*t9.*t11.*(-1.0./2.0);
t1483 = Iyz6.*t3.*t4.*t12.*t13.*(-1.0./2.0);
t1484 = Iyz6.*t3.*t7.*t10.*t12.*(-1.0./2.0);
t1485 = Iyz6.*t4.*t7.*t9.*t12.*(-1.0./2.0);
t1486 = Izy5.*t3.*t6.*t10.*t11.*(-1.0./2.0);
t1487 = Izy5.*t4.*t6.*t9.*t11.*(-1.0./2.0);
t1488 = Izy6.*t3.*t4.*t11.*t13.*(-1.0./2.0);
t1489 = Izy6.*t3.*t7.*t10.*t11.*(-1.0./2.0);
t1490 = Izy6.*t4.*t7.*t9.*t11.*(-1.0./2.0);
t1491 = Izy6.*t3.*t4.*t12.*t13.*(-1.0./2.0);
M = ft_1({Ixx2,Ixx3,Ixx4,Ixx5,Ixx6,Ixy4,Ixy5,Ixy6,Ixz2,Ixz3,Ixz4,Ixz5,Ixz6,Iyx4,Iyx5,Iyx6,Iyy2,Iyy3,Iyy4,Iyy5,Iyy6,Iyz4,Iyz5,Iyz6,Izx2,Izx3,Izx4,Izx5,Izx6,Izy4,Izy5,Izy6,Izz1,Izz2,Izz3,Izz4,Izz5,Izz6,Lx3,Lxcm1,Lxcm2,Lxcm3,Lxcm4,Lxcm5,Lxcm6,Lycm1,Lycm2,Lycm3,Lycm4,Lycm5,Lycm6,Lz4,Lz5,Lzcm2,Lzcm3,Lzcm4,Lzcm5,Lzcm6,m1,m2,m3,m4,m5,m6,t10,t100,t1023,t1037,t1038,t1040,t1041,t1049,t1050,t1054,t1057,t1058,t1062,t1067,t1072,t1095,t1096,t1097,t1098,t1099,t11,t1100,t111,t112,t1124,t1125,t113,t1132,t1134,t1136,t1137,t114,t115,t116,t1169,t117,t1170,t118,t1180,t1181,t1191,t1193,t12,t1205,t1207,t126,t127,t128,t1286,t129,t13,t130,t131,t1311,t1312,t1315,t1316,t1317,t132,t133,t134,t1344,t135,t1354,t136,t137,t138,t139,t140,t141,t142,t143,t144,t145,t1466,t1467,t147,t1472,t1473,t1478,t1479,t1480,t1481,t1482,t1483,t1484,t1485,t1486,t1487,t1488,t1489,t149,t1490,t1491,t15,t150,t151,t152,t153,t154,t155,t18,t2,t203,t204,t205,t206,t207,t210,t214,t215,t216,t217,t218,t219,t220,t221,t222,t223,t224,t225,t226,t227,t228,t229,t230,t231,t232,t233,t234,t235,t236,t237,t238,t240,t242,t243,t244,t245,t246,t247,t248,t249,t250,t251,t252,t254,t256,t258,t260,t261,t262,t263,t264,t265,t266,t267,t268,t269,t270,t271,t272,t274,t276,t277,t278,t279,t280,t281,t282,t283,t284,t285,t286,t287,t288,t289,t290,t299,t3,t303,t307,t308,t309,t310,t312,t314,t316,t318,t319,t320,t321,t322,t324,t326,t328,t33,t330,t331,t332,t333,t334,t335,t336,t337,t338,t34,t35,t36,t366,t367,t37,t371,t372,t379,t38,t380,t381,t383,t384,t385,t387,t388,t389,t39,t393,t394,t395,t399,t4,t40,t400,t401,t41,t42,t43,t44,t441,t442,t444,t445,t45,t454,t455,t456,t457,t458,t459,t46,t460,t461,t462,t463,t464,t465,t466,t467,t468,t469,t47,t470,t472,t473,t475,t476,t477,t478,t48,t481,t482,t485,t486,t49,t490,t495,t496,t498,t499,t5,t50,t502,t503,t507,t508,t509,t51,t513,t514,t515,t516,t517,t518,t519,t52,t520,t521,t522,t523,t524,t525,t526,t528,t529,t53,t530,t531,t532,t533,t534,t535,t536,t537,t539,t54,t543,t544,t546,t547,t55,t551,t552,t553,t554,t555,t556,t557,t558,t559,t56,t560,t563,t564,t565,t566,t567,t568,t57,t58,t59,t6,t60,t61,t62,t63,t637,t64,t65,t66,t661,t669,t67,t670,t68,t69,t698,t699,t7,t70,t701,t702,t704,t705,t707,t708,t71,t712,t713,t715,t716,t718,t719,t72,t721,t722,t725,t726,t728,t729,t73,t733,t734,t736,t737,t74,t75,t76,t765,t77,t778,t779,t78,t780,t781,t79,t793,t795,t797,t798,t8,t80,t800,t802,t803,t805,t806,t81,t810,t811,t815,t816,t818,t819,t82,t821,t822,t824,t825,t829,t83,t830,t834,t838,t839,t84,t840,t841,t843,t844,t848,t849,t85,t850,t851,t854,t856,t86,t868,t87,t870,t877,t878,t879,t88,t880,t882,t883,t884,t885,t887,t888,t889,t89,t890,t891,t892,t893,t895,t896,t897,t899,t9,t90,t900,t901,t902,t91,t914,t918,t919,t92,t920,t925,t926,t927,t93,t94,t95,t951,t952,t96,t97,t98,t99});
end
function out1 = ft_1(ct)
[Ixx2,Ixx3,Ixx4,Ixx5,Ixx6,Ixy4,Ixy5,Ixy6,Ixz2,Ixz3,Ixz4,Ixz5,Ixz6,Iyx4,Iyx5,Iyx6,Iyy2,Iyy3,Iyy4,Iyy5,Iyy6,Iyz4,Iyz5,Iyz6,Izx2,Izx3,Izx4,Izx5,Izx6,Izy4,Izy5,Izy6,Izz1,Izz2,Izz3,Izz4,Izz5,Izz6,Lx3,Lxcm1,Lxcm2,Lxcm3,Lxcm4,Lxcm5,Lxcm6,Lycm1,Lycm2,Lycm3,Lycm4,Lycm5,Lycm6,Lz4,Lz5,Lzcm2,Lzcm3,Lzcm4,Lzcm5,Lzcm6,m1,m2,m3,m4,m5,m6,t10,t100,t1023,t1037,t1038,t1040,t1041,t1049,t1050,t1054,t1057,t1058,t1062,t1067,t1072,t1095,t1096,t1097,t1098,t1099,t11,t1100,t111,t112,t1124,t1125,t113,t1132,t1134,t1136,t1137,t114,t115,t116,t1169,t117,t1170,t118,t1180,t1181,t1191,t1193,t12,t1205,t1207,t126,t127,t128,t1286,t129,t13,t130,t131,t1311,t1312,t1315,t1316,t1317,t132,t133,t134,t1344,t135,t1354,t136,t137,t138,t139,t140,t141,t142,t143,t144,t145,t1466,t1467,t147,t1472,t1473,t1478,t1479,t1480,t1481,t1482,t1483,t1484,t1485,t1486,t1487,t1488,t1489,t149,t1490,t1491,t15,t150,t151,t152,t153,t154,t155,t18,t2,t203,t204,t205,t206,t207,t210,t214,t215,t216,t217,t218,t219,t220,t221,t222,t223,t224,t225,t226,t227,t228,t229,t230,t231,t232,t233,t234,t235,t236,t237,t238,t240,t242,t243,t244,t245,t246,t247,t248,t249,t250,t251,t252,t254,t256,t258,t260,t261,t262,t263,t264,t265,t266,t267,t268,t269,t270,t271,t272,t274,t276,t277,t278,t279,t280,t281,t282,t283,t284,t285,t286,t287,t288,t289,t290,t299,t3,t303,t307,t308,t309,t310,t312,t314,t316,t318,t319,t320,t321,t322,t324,t326,t328,t33,t330,t331,t332,t333,t334,t335,t336,t337,t338,t34,t35,t36,t366,t367,t37,t371,t372,t379,t38,t380,t381,t383,t384,t385,t387,t388,t389,t39,t393,t394,t395,t399,t4,t40,t400,t401,t41,t42,t43,t44,t441,t442,t444,t445,t45,t454,t455,t456,t457,t458,t459,t46,t460,t461,t462,t463,t464,t465,t466,t467,t468,t469,t47,t470,t472,t473,t475,t476,t477,t478,t48,t481,t482,t485,t486,t49,t490,t495,t496,t498,t499,t5,t50,t502,t503,t507,t508,t509,t51,t513,t514,t515,t516,t517,t518,t519,t52,t520,t521,t522,t523,t524,t525,t526,t528,t529,t53,t530,t531,t532,t533,t534,t535,t536,t537,t539,t54,t543,t544,t546,t547,t55,t551,t552,t553,t554,t555,t556,t557,t558,t559,t56,t560,t563,t564,t565,t566,t567,t568,t57,t58,t59,t6,t60,t61,t62,t63,t637,t64,t65,t66,t661,t669,t67,t670,t68,t69,t698,t699,t7,t70,t701,t702,t704,t705,t707,t708,t71,t712,t713,t715,t716,t718,t719,t72,t721,t722,t725,t726,t728,t729,t73,t733,t734,t736,t737,t74,t75,t76,t765,t77,t778,t779,t78,t780,t781,t79,t793,t795,t797,t798,t8,t80,t800,t802,t803,t805,t806,t81,t810,t811,t815,t816,t818,t819,t82,t821,t822,t824,t825,t829,t83,t830,t834,t838,t839,t84,t840,t841,t843,t844,t848,t849,t85,t850,t851,t854,t856,t86,t868,t87,t870,t877,t878,t879,t88,t880,t882,t883,t884,t885,t887,t888,t889,t89,t890,t891,t892,t893,t895,t896,t897,t899,t9,t90,t900,t901,t902,t91,t914,t918,t919,t92,t920,t925,t926,t927,t93,t94,t95,t951,t952,t96,t97,t98,t99] = ct{:};
t1492 = Izy6.*t3.*t7.*t10.*t12.*(-1.0./2.0);
t1493 = Izy6.*t4.*t7.*t9.*t12.*(-1.0./2.0);
t1509 = Ixy6.*t3.*t10.*t11.*t12.*(-1.0./2.0);
t1510 = Ixy6.*t4.*t9.*t11.*t12.*(-1.0./2.0);
t1511 = Ixz6.*t3.*t10.*t11.*t13.*(-1.0./2.0);
t1512 = Ixz6.*t4.*t9.*t11.*t13.*(-1.0./2.0);
t1513 = Ixz6.*t7.*t9.*t10.*t11.*(-1.0./2.0);
t1514 = Ixz6.*t3.*t10.*t12.*t13.*(-1.0./2.0);
t1515 = Ixz6.*t4.*t9.*t12.*t13.*(-1.0./2.0);
t1516 = Ixz6.*t7.*t9.*t10.*t12.*(-1.0./2.0);
t1518 = Iyx6.*t3.*t10.*t11.*t12.*(-1.0./2.0);
t1519 = Iyx6.*t4.*t9.*t11.*t12.*(-1.0./2.0);
t1520 = Izx6.*t3.*t10.*t11.*t13.*(-1.0./2.0);
t1521 = Izx6.*t4.*t9.*t11.*t13.*(-1.0./2.0);
t1522 = Izx6.*t7.*t9.*t10.*t11.*(-1.0./2.0);
t1523 = Izx6.*t3.*t10.*t12.*t13.*(-1.0./2.0);
t1524 = Izx6.*t4.*t9.*t12.*t13.*(-1.0./2.0);
t1525 = Izx6.*t7.*t9.*t10.*t12.*(-1.0./2.0);
t1610 = Lxcm6.*Lycm6.*m6.*t3.*t7.*t10.*t11.*t13.*2.0;
t1611 = Lxcm6.*Lycm6.*m6.*t4.*t7.*t9.*t11.*t13.*2.0;
t1782 = Iyz6.*t3.*t5.*t6.*t10.*t13.*(-1.0./2.0);
t1784 = Iyz6.*t4.*t5.*t6.*t9.*t13.*(-1.0./2.0);
t1786 = Izy6.*t3.*t5.*t6.*t10.*t13.*(-1.0./2.0);
t1788 = Izy6.*t4.*t5.*t6.*t9.*t13.*(-1.0./2.0);
t1986 = Lxcm6.*Lycm6.*m6.*t3.*t5.*t7.*t10.*t11.*t13.*-2.0;
t1987 = Lxcm6.*Lycm6.*m6.*t4.*t5.*t7.*t9.*t11.*t13.*-2.0;
t101 = Ixx4.*t34;
t102 = Ixx5.*t35;
t103 = Ixx6.*t34;
t104 = Iyy4.*t34;
t105 = Iyy5.*t34;
t106 = Iyy6.*t35;
t107 = Izz5.*t34;
t108 = Izz5.*t35;
t109 = Izz6.*t34;
t110 = Izz6.*t35;
t119 = t5.*t50;
t120 = t6.*t51;
t121 = t5.*t54;
t122 = t6.*t54;
t123 = t5.*t57;
t124 = t5.*t60;
t125 = t5.*t61;
t146 = t6.*t43;
t148 = t12.*t43;
t156 = -t62;
t157 = -t65;
t158 = -t75;
t159 = -t76;
t160 = -t77;
t161 = -t78;
t162 = -t79;
t163 = -t80;
t164 = -t116;
t165 = -t117;
t166 = -t85;
t167 = -t118;
t168 = -t93;
t169 = -t94;
t170 = -t96;
t171 = -t97;
t172 = -t98;
t173 = -t99;
t174 = -t126;
t175 = -t127;
t176 = -t128;
t177 = -t129;
t178 = -t130;
t179 = -t131;
t180 = -t132;
t181 = -t133;
t182 = -t136;
t183 = -t137;
t184 = -t139;
t185 = -t142;
t186 = -t143;
t187 = -t145;
t188 = t36.*t40;
t189 = Iyy6.*t5.*t36;
t190 = Ixy6.*t12.*t36;
t191 = Ixz5.*t11.*t35;
t192 = Iyx6.*t12.*t36;
t193 = Izx5.*t11.*t35;
t194 = Lxcm4.*Lycm4.*m4.*t37;
t195 = Lxcm6.*Lycm6.*m6.*t39;
t196 = Lxcm5.*Lzcm5.*m5.*t38;
t202 = t3.*t4.*t42;
t208 = t5.*t76;
t209 = t6.*t76;
t211 = t5.*t79;
t212 = t5.*t80;
t213 = t6.*t80;
t239 = t5.*t84;
t241 = t5.*t85;
t253 = t5.*t93;
t255 = t6.*t93;
t257 = t5.*t96;
t259 = t6.*t96;
t273 = t9.*t10.*t42;
t275 = t11.*t12.*t42;
t291 = t9.*t10.*t51;
t292 = t11.*t12.*t51;
t293 = t9.*t10.*t52;
t294 = t9.*t10.*t53;
t295 = t11.*t12.*t54;
t296 = t9.*t10.*t57;
t297 = t9.*t10.*t60;
t298 = t9.*t10.*t61;
t300 = t5.*t128;
t301 = t5.*t129;
t302 = t6.*t129;
t304 = t5.*t132;
t305 = t5.*t133;
t306 = t6.*t133;
t311 = t5.*t135;
t313 = t5.*t136;
t315 = t5.*t139;
t317 = t6.*t139;
t323 = t5.*t141;
t325 = t5.*t142;
t327 = t5.*t145;
t329 = t6.*t145;
t339 = t5.*t6.*t44;
t340 = t5.*t12.*t44;
t341 = t7.*t11.*t44;
t342 = t11.*t13.*t44;
t343 = t34.*t45;
t344 = t35.*t45;
t345 = m4.*t18.*t34;
t346 = t35.*t50;
t347 = t34.*t51;
t348 = t34.*t52;
t349 = t34.*t53;
t350 = t35.*t54;
t351 = t34.*t57;
t352 = t35.*t57;
t353 = t34.*t60;
t354 = t35.*t60;
t355 = t34.*t61;
t356 = t35.*t61;
t357 = -t152;
t358 = -t155;
t359 = (Ixy4.*t37)./2.0;
t360 = (Ixy6.*t39)./2.0;
t361 = (Ixz5.*t38)./2.0;
t362 = (Iyx4.*t37)./2.0;
t363 = (Iyx6.*t39)./2.0;
t364 = (Izx5.*t38)./2.0;
t365 = t5.*t74.*2.0;
t368 = t5.*t88.*2.0;
t369 = t5.*t91.*2.0;
t370 = t5.*t92.*2.0;
t373 = t3.*t4.*t51;
t374 = t3.*t4.*t52;
t375 = t3.*t4.*t53;
t376 = t3.*t4.*t57;
t377 = t3.*t4.*t60;
t378 = t3.*t4.*t61;
t382 = -t299;
t386 = -t303;
t390 = -t309;
t391 = -t310;
t392 = -t312;
t396 = -t321;
t397 = -t322;
t398 = -t324;
t402 = t35.*t66;
t403 = Ixx6.*t3.*t4.*t36;
t404 = t35.*t67;
t405 = t36.*t67;
t408 = -t332;
t409 = -t333;
t410 = -t334;
t411 = -t336;
t412 = -t337;
t413 = -t338;
t414 = Ixy4.*t3.*t10.*t34;
t415 = Ixy4.*t4.*t9.*t34;
t417 = Ixy6.*t6.*t11.*t36;
t418 = Ixy6.*t7.*t13.*t34;
t419 = Ixy6.*t7.*t13.*t35;
t420 = Ixz5.*t6.*t12.*t34;
t421 = Ixz6.*t7.*t11.*t35;
t422 = Iyx4.*t3.*t10.*t34;
t423 = Iyx4.*t4.*t9.*t34;
t425 = Iyx6.*t6.*t11.*t36;
t426 = Iyx6.*t7.*t13.*t34;
t427 = Iyx6.*t7.*t13.*t35;
t428 = Izx5.*t6.*t12.*t34;
t429 = Izx6.*t7.*t11.*t35;
t430 = t35.*t97;
t431 = Ixx6.*t9.*t10.*t36;
t432 = t35.*t98;
t433 = t36.*t98;
t434 = Iyz6.*t11.*t13.*t35;
t435 = Izy6.*t11.*t13.*t35;
t443 = t5.*t205;
t447 = t6.*t207;
t471 = t3.*t4.*t84;
t474 = t3.*t4.*t85;
t479 = t5.*t243;
t480 = t5.*t244;
t483 = t5.*t245;
t484 = t5.*t246;
t487 = t5.*t247;
t488 = t5.*t248;
t489 = t6.*t251;
t491 = t6.*t252;
t493 = t6.*t254;
t497 = t3.*t4.*t95;
t501 = t6.*t258;
t504 = t3.*t10.*t11.*t40;
t505 = t4.*t9.*t11.*t40;
t506 = t7.*t12.*t13.*t40;
t510 = t3.*t10.*t11.*t41;
t511 = t4.*t9.*t11.*t41;
t512 = t5.*t268;
t527 = t5.*t278;
t538 = t9.*t10.*t75;
t540 = t6.*t280;
t541 = t6.*t281;
t545 = t9.*t10.*t78;
t548 = t9.*t10.*t79;
t549 = t6.*t285;
t561 = t9.*t10.*t84;
t562 = t9.*t10.*t85;
t570 = t9.*t10.*t94;
t571 = t9.*t10.*t95;
t577 = -t207;
t580 = -t210;
t586 = Ixx6.*t35.*t36;
t588 = Iyy6.*t34.*t36;
t592 = -t217;
t593 = -t219;
t594 = -t220;
t595 = -t221;
t596 = -t223;
t597 = -t224;
t598 = -t225;
t599 = -t227;
t600 = -t228;
t601 = -t229;
t602 = -t231;
t603 = -t232;
t604 = -t233;
t605 = -t367;
t606 = -t234;
t607 = -t237;
t608 = -t238;
t609 = -t240;
t611 = -t249;
t612 = -t250;
t613 = -t251;
t614 = -t252;
t616 = -t371;
t620 = -t263;
t621 = -t264;
t622 = -t267;
t623 = -t269;
t624 = -t271;
t626 = -t277;
t627 = -t278;
t628 = -t379;
t629 = -t279;
t630 = -t281;
t631 = -t282;
t632 = -t284;
t633 = -t285;
t634 = -t286;
t635 = -t287;
t636 = -t288;
t638 = -t289;
t639 = -t290;
t646 = t36.*t85.*2.0;
t647 = t35.*t95.*2.0;
t648 = t5.*t36.*t51;
t652 = t5.*t206.*2.0;
t658 = t5.*t233.*2.0;
t659 = t5.*t240.*2.0;
t660 = t5.*t242.*2.0;
t662 = t6.*t256.*2.0;
t663 = t6.*t260.*2.0;
t666 = t6.*t282.*2.0;
t667 = t5.*t284.*2.0;
t668 = t6.*t286.*2.0;
t672 = t3.*t10.*t11.*t50;
t673 = t4.*t9.*t11.*t50;
t675 = t6.*t11.*t12.*t50;
t676 = t7.*t12.*t13.*t51;
t677 = t3.*t10.*t11.*t54;
t678 = t4.*t9.*t11.*t54;
t681 = t7.*t12.*t13.*t54;
t682 = t3.*t10.*t11.*t57;
t683 = t4.*t9.*t11.*t57;
t684 = t6.*t11.*t12.*t57;
t685 = t3.*t10.*t11.*t60;
t686 = t4.*t9.*t11.*t60;
t687 = t3.*t10.*t11.*t61;
t688 = t4.*t9.*t11.*t61;
t689 = t6.*t11.*t12.*t60;
t690 = t6.*t11.*t12.*t61;
t697 = t3.*t4.*t135;
t706 = t3.*t4.*t138;
t711 = t3.*t4.*t141;
t720 = t3.*t4.*t144;
t727 = t9.*t10.*t127;
t730 = t9.*t10.*t128;
t731 = t6.*t333;
t735 = t9.*t10.*t131;
t738 = t9.*t10.*t132;
t739 = t6.*t337;
t742 = t9.*t10.*t136;
t743 = t9.*t10.*t137;
t747 = t9.*t10.*t142;
t748 = t9.*t10.*t143;
t764 = t3.*t4.*t5.*t74;
t766 = t6.*t444;
t767 = t5.*t445;
t773 = t3.*t4.*t220;
t774 = t3.*t4.*t224;
t782 = t6.*t464;
t783 = t6.*t465;
t784 = t5.*t469;
t785 = t6.*t468;
t787 = t5.*t472;
t788 = t5.*t473;
t790 = t5.*t475;
t791 = t5.*t476;
t792 = t3.*t4.*t5.*t88;
t794 = t3.*t4.*t5.*t91;
t799 = t3.*t4.*t5.*t92;
t804 = t3.*t4.*t254;
t808 = t3.*t4.*t256;
t809 = t3.*t4.*t258;
t813 = t3.*t4.*t260;
t814 = t6.*t11.*t12.*t66;
t820 = t6.*t11.*t12.*t67;
t823 = t7.*t12.*t13.*t67;
t826 = t3.*t4.*t270;
t827 = t3.*t4.*t272;
t828 = t3.*t4.*t274;
t832 = t3.*t5.*t10.*t12.*t42;
t833 = t4.*t5.*t9.*t12.*t42;
t835 = t3.*t10.*t11.*t74;
t836 = t4.*t9.*t11.*t74;
t837 = t5.*t9.*t10.*t74;
t842 = t6.*t529;
t845 = t6.*t532;
t846 = t5.*t535;
t847 = t6.*t533;
t852 = t9.*t10.*t207;
t853 = t3.*t4.*t281;
t858 = t3.*t4.*t282;
t859 = t3.*t10.*t12.*t76;
t860 = t4.*t9.*t12.*t76;
t862 = t5.*t546;
t864 = t5.*t547;
t867 = t3.*t4.*t285;
t872 = t3.*t4.*t286;
t873 = t3.*t10.*t12.*t80;
t874 = t4.*t9.*t12.*t80;
t903 = t5.*t560;
t904 = t6.*t559;
t905 = t3.*t10.*t11.*t84;
t906 = t4.*t9.*t11.*t84;
t911 = t3.*t10.*t11.*t88;
t912 = t4.*t9.*t11.*t88;
t913 = t5.*t9.*t10.*t88;
t915 = t3.*t10.*t11.*t91;
t916 = t4.*t9.*t11.*t91;
t917 = t5.*t9.*t10.*t91;
t921 = t9.*t10.*t250;
t922 = t3.*t10.*t11.*t92;
t923 = t4.*t9.*t11.*t92;
t924 = t5.*t9.*t10.*t92;
t928 = t9.*t10.*t251;
t931 = t9.*t10.*t254;
t932 = t3.*t10.*t12.*t93;
t933 = t4.*t9.*t12.*t93;
t935 = t9.*t10.*t256;
t938 = t9.*t10.*t258;
t939 = t3.*t10.*t12.*t96;
t940 = t4.*t9.*t12.*t96;
t942 = t9.*t10.*t260;
t943 = t6.*t11.*t12.*t97;
t944 = t9.*t10.*t264;
t945 = t6.*t11.*t12.*t98;
t947 = t9.*t10.*t270;
t948 = t9.*t10.*t272;
t949 = t9.*t10.*t274;
t953 = t9.*t10.*t281;
t954 = t9.*t10.*t282;
t955 = t9.*t10.*t285;
t956 = t9.*t10.*t286;
t957 = t9.*t10.*t287;
t958 = t9.*t10.*t288;
t959 = t9.*t10.*t289;
t966 = -t458;
t967 = -t461;
t968 = -t464;
t969 = -t465;
t970 = -t467;
t971 = -t468;
t972 = -t469;
t973 = -t470;
t975 = -t472;
t976 = -t473;
t979 = -t661;
t981 = -t490;
t987 = -t498;
t988 = -t499;
t992 = -t502;
t993 = -t503;
t995 = -t513;
t996 = -t514;
t997 = -t515;
t998 = -t516;
t999 = -t517;
t1000 = -t518;
t1001 = -t519;
t1002 = -t520;
t1003 = -t521;
t1004 = -t524;
t1005 = -t525;
t1007 = -t528;
t1008 = -t529;
t1009 = -t531;
t1010 = -t532;
t1011 = -t533;
t1012 = -t534;
t1013 = -t535;
t1014 = -t536;
t1015 = -t537;
t1017 = -t543;
t1018 = -t544;
t1019 = -t546;
t1020 = -t547;
t1024 = -t551;
t1025 = -t552;
t1026 = -t553;
t1027 = -t554;
t1028 = -t555;
t1029 = -t556;
t1031 = -t564;
t1032 = -t566;
t1033 = -t568;
t1039 = t6.*t384;
t1042 = t6.*t388;
t1047 = -t698;
t1048 = -t699;
t1051 = -t707;
t1052 = -t708;
t1053 = t6.*t394;
t1055 = -t712;
t1056 = -t713;
t1059 = -t721;
t1060 = -t722;
t1061 = t6.*t400;
t1063 = -t725;
t1064 = -t726;
t1065 = -t728;
t1066 = -t729;
t1068 = -t733;
t1069 = -t734;
t1070 = -t736;
t1071 = -t737;
t1073 = Ixy5.*t3.*t6.*t10.*t34;
t1074 = Ixy5.*t4.*t6.*t9.*t34;
t1075 = Ixy6.*t3.*t6.*t10.*t34;
t1076 = Ixy6.*t4.*t6.*t9.*t34;
t1078 = Ixy6.*t3.*t6.*t10.*t36;
t1079 = Ixy6.*t4.*t6.*t9.*t36;
t1081 = Ixz5.*t3.*t5.*t10.*t35;
t1082 = Ixz5.*t4.*t5.*t9.*t35;
t1083 = t34.*t220;
t1084 = Iyx5.*t3.*t6.*t10.*t34;
t1085 = Iyx5.*t4.*t6.*t9.*t34;
t1086 = Iyx6.*t3.*t6.*t10.*t34;
t1087 = Iyx6.*t4.*t6.*t9.*t34;
t1089 = Iyx6.*t3.*t6.*t10.*t36;
t1090 = Iyx6.*t4.*t6.*t9.*t36;
t1092 = Izx5.*t3.*t5.*t10.*t35;
t1093 = Izx5.*t4.*t5.*t9.*t35;
t1094 = t34.*t224;
t1101 = t36.*t261;
t1102 = t36.*t262;
t1103 = Ixx6.*t6.*t11.*t12.*t36;
t1104 = Iyy6.*t3.*t10.*t11.*t36;
t1105 = Iyy6.*t4.*t9.*t11.*t36;
t1106 = t36.*t267;
t1107 = Iyz5.*t3.*t10.*t12.*t34;
t1108 = Iyz5.*t4.*t9.*t12.*t34;
t1109 = t34.*t270;
t1110 = Izy5.*t3.*t10.*t12.*t34;
t1111 = Izy5.*t4.*t9.*t12.*t34;
t1112 = t34.*t272;
t1113 = t35.*t281.*2.0;
t1114 = t35.*t285.*2.0;
t1119 = t9.*t10.*t36.*t54;
t1126 = t6.*t7.*t11.*t13.*t40.*2.0;
out1 = ft_2({Ixx2,Ixx3,Ixx4,Ixx5,Ixx6,Ixy4,Ixy5,Ixy6,Ixz2,Ixz3,Ixz4,Ixz5,Ixz6,Iyx4,Iyx5,Iyx6,Iyy2,Iyy3,Iyy4,Iyy5,Iyy6,Iyz4,Iyz5,Iyz6,Izx2,Izx3,Izx4,Izx5,Izx6,Izy4,Izy5,Izy6,Izz1,Izz2,Izz3,Izz4,Izz5,Izz6,Lx3,Lxcm1,Lxcm2,Lxcm3,Lxcm4,Lxcm5,Lxcm6,Lycm1,Lycm2,Lycm3,Lycm4,Lycm5,Lycm6,Lz4,Lz5,Lzcm2,Lzcm3,Lzcm4,Lzcm5,Lzcm6,m1,m2,m3,m4,m5,m6,t10,t100,t1000,t1001,t1002,t1003,t1004,t1005,t1007,t1008,t1009,t101,t1010,t1011,t1012,t1013,t1014,t1015,t1017,t1018,t1019,t102,t1020,t1023,t1024,t1025,t1026,t1027,t1028,t1029,t103,t1031,t1032,t1033,t1037,t1038,t1039,t104,t1040,t1041,t1042,t1047,t1048,t1049,t105,t1050,t1051,t1052,t1053,t1054,t1055,t1056,t1057,t1058,t1059,t106,t1060,t1061,t1062,t1063,t1064,t1065,t1066,t1067,t1068,t1069,t107,t1070,t1071,t1072,t1073,t1074,t1075,t1076,t1078,t1079,t108,t1081,t1082,t1083,t1084,t1085,t1086,t1087,t1089,t109,t1090,t1092,t1093,t1094,t1095,t1096,t1097,t1098,t1099,t11,t110,t1100,t1101,t1102,t1103,t1104,t1105,t1106,t1107,t1108,t1109,t111,t1110,t1111,t1112,t1113,t1114,t1119,t112,t1124,t1125,t1126,t113,t1132,t1134,t1136,t1137,t114,t115,t1169,t1170,t1180,t1181,t119,t1191,t1193,t12,t120,t1205,t1207,t121,t122,t123,t124,t125,t1286,t13,t1311,t1312,t1315,t1316,t1317,t134,t1344,t135,t1354,t138,t140,t141,t144,t146,t1466,t1467,t147,t1472,t1473,t1478,t1479,t148,t1480,t1481,t1482,t1483,t1484,t1485,t1486,t1487,t1488,t1489,t149,t1490,t1491,t1492,t1493,t15,t150,t1509,t151,t1510,t1511,t1512,t1513,t1514,t1515,t1516,t1518,t1519,t1520,t1521,t1522,t1523,t1524,t1525,t153,t154,t156,t157,t158,t159,t160,t161,t1610,t1611,t162,t163,t164,t165,t166,t167,t168,t169,t170,t171,t172,t173,t174,t175,t176,t177,t178,t1782,t1784,t1786,t1788,t179,t18,t180,t181,t182,t183,t184,t185,t186,t187,t188,t189,t190,t191,t192,t193,t194,t195,t196,t1986,t1987,t2,t202,t203,t204,t205,t206,t208,t209,t211,t212,t213,t214,t215,t216,t218,t219,t220,t222,t223,t224,t226,t227,t230,t231,t233,t235,t236,t237,t238,t239,t241,t242,t243,t244,t245,t246,t247,t248,t253,t254,t255,t256,t257,t258,t259,t260,t261,t262,t265,t266,t268,t270,t272,t273,t274,t275,t276,t278,t280,t282,t283,t286,t291,t292,t293,t294,t295,t296,t297,t298,t3,t300,t301,t302,t304,t305,t306,t307,t308,t311,t313,t314,t315,t316,t317,t318,t319,t320,t323,t325,t326,t327,t328,t329,t33,t330,t331,t333,t334,t335,t337,t338,t339,t34,t340,t341,t342,t343,t344,t345,t346,t347,t348,t349,t35,t350,t351,t352,t353,t354,t355,t356,t357,t358,t359,t36,t360,t361,t362,t363,t364,t365,t366,t368,t369,t370,t372,t373,t374,t375,t376,t377,t378,t380,t381,t382,t383,t384,t385,t386,t387,t388,t389,t390,t391,t392,t393,t394,t395,t396,t397,t398,t399,t4,t40,t400,t401,t402,t403,t404,t405,t408,t409,t41,t410,t411,t412,t413,t414,t415,t417,t418,t419,t42,t420,t421,t422,t423,t425,t426,t427,t428,t429,t43,t430,t431,t432,t433,t434,t435,t44,t441,t442,t443,t444,t445,t447,t45,t454,t455,t456,t457,t459,t46,t460,t462,t463,t466,t467,t47,t471,t472,t473,t474,t475,t476,t477,t478,t479,t48,t480,t481,t482,t483,t484,t485,t486,t487,t488,t489,t49,t491,t493,t495,t496,t497,t498,t499,t5,t50,t501,t504,t505,t506,t507,t508,t509,t51,t510,t511,t512,t513,t52,t522,t523,t526,t527,t53,t530,t531,t535,t538,t539,t54,t540,t541,t545,t546,t547,t548,t549,t55,t551,t554,t557,t558,t559,t56,t560,t561,t562,t563,t565,t567,t57,t570,t571,t577,t58,t580,t586,t588,t59,t592,t593,t594,t595,t596,t597,t598,t599,t6,t60,t600,t601,t602,t603,t604,t605,t606,t607,t608,t609,t61,t611,t612,t613,t614,t616,t62,t620,t621,t622,t623,t624,t626,t627,t628,t629,t63,t630,t631,t632,t633,t634,t635,t636,t637,t638,t639,t64,t646,t647,t648,t65,t652,t658,t659,t66,t660,t662,t663,t666,t667,t668,t669,t67,t670,t672,t673,t675,t676,t677,t678,t68,t681,t682,t683,t684,t685,t686,t687,t688,t689,t69,t690,t697,t698,t699,t7,t70,t701,t702,t704,t705,t706,t71,t711,t712,t713,t715,t716,t718,t719,t72,t720,t727,t728,t729,t73,t730,t731,t735,t736,t737,t738,t739,t74,t742,t743,t747,t748,t764,t765,t766,t767,t773,t774,t778,t779,t780,t781,t782,t783,t784,t785,t787,t788,t790,t791,t792,t793,t794,t795,t797,t798,t799,t8,t800,t802,t803,t804,t805,t806,t808,t809,t81,t810,t811,t813,t814,t815,t816,t818,t819,t82,t820,t821,t822,t823,t824,t825,t826,t827,t828,t829,t83,t830,t832,t833,t834,t835,t836,t837,t838,t839,t84,t840,t841,t842,t843,t844,t845,t846,t847,t848,t849,t85,t850,t851,t852,t853,t854,t856,t858,t859,t86,t860,t862,t864,t867,t868,t87,t870,t872,t873,t874,t877,t878,t879,t88,t880,t882,t883,t884,t885,t887,t888,t889,t89,t890,t891,t892,t893,t895,t896,t897,t899,t9,t90,t900,t901,t902,t903,t904,t905,t906,t91,t911,t912,t913,t914,t915,t916,t917,t918,t919,t92,t920,t921,t922,t923,t924,t925,t926,t927,t928,t931,t932,t933,t935,t938,t939,t940,t942,t943,t944,t945,t947,t948,t949,t95,t951,t952,t953,t954,t955,t956,t957,t958,t959,t966,t967,t968,t969,t970,t971,t972,t973,t975,t976,t979,t981,t987,t988,t992,t993,t995,t996,t997,t998,t999});
end
function out1 = ft_2(ct)
[Ixx2,Ixx3,Ixx4,Ixx5,Ixx6,Ixy4,Ixy5,Ixy6,Ixz2,Ixz3,Ixz4,Ixz5,Ixz6,Iyx4,Iyx5,Iyx6,Iyy2,Iyy3,Iyy4,Iyy5,Iyy6,Iyz4,Iyz5,Iyz6,Izx2,Izx3,Izx4,Izx5,Izx6,Izy4,Izy5,Izy6,Izz1,Izz2,Izz3,Izz4,Izz5,Izz6,Lx3,Lxcm1,Lxcm2,Lxcm3,Lxcm4,Lxcm5,Lxcm6,Lycm1,Lycm2,Lycm3,Lycm4,Lycm5,Lycm6,Lz4,Lz5,Lzcm2,Lzcm3,Lzcm4,Lzcm5,Lzcm6,m1,m2,m3,m4,m5,m6,t10,t100,t1000,t1001,t1002,t1003,t1004,t1005,t1007,t1008,t1009,t101,t1010,t1011,t1012,t1013,t1014,t1015,t1017,t1018,t1019,t102,t1020,t1023,t1024,t1025,t1026,t1027,t1028,t1029,t103,t1031,t1032,t1033,t1037,t1038,t1039,t104,t1040,t1041,t1042,t1047,t1048,t1049,t105,t1050,t1051,t1052,t1053,t1054,t1055,t1056,t1057,t1058,t1059,t106,t1060,t1061,t1062,t1063,t1064,t1065,t1066,t1067,t1068,t1069,t107,t1070,t1071,t1072,t1073,t1074,t1075,t1076,t1078,t1079,t108,t1081,t1082,t1083,t1084,t1085,t1086,t1087,t1089,t109,t1090,t1092,t1093,t1094,t1095,t1096,t1097,t1098,t1099,t11,t110,t1100,t1101,t1102,t1103,t1104,t1105,t1106,t1107,t1108,t1109,t111,t1110,t1111,t1112,t1113,t1114,t1119,t112,t1124,t1125,t1126,t113,t1132,t1134,t1136,t1137,t114,t115,t1169,t1170,t1180,t1181,t119,t1191,t1193,t12,t120,t1205,t1207,t121,t122,t123,t124,t125,t1286,t13,t1311,t1312,t1315,t1316,t1317,t134,t1344,t135,t1354,t138,t140,t141,t144,t146,t1466,t1467,t147,t1472,t1473,t1478,t1479,t148,t1480,t1481,t1482,t1483,t1484,t1485,t1486,t1487,t1488,t1489,t149,t1490,t1491,t1492,t1493,t15,t150,t1509,t151,t1510,t1511,t1512,t1513,t1514,t1515,t1516,t1518,t1519,t1520,t1521,t1522,t1523,t1524,t1525,t153,t154,t156,t157,t158,t159,t160,t161,t1610,t1611,t162,t163,t164,t165,t166,t167,t168,t169,t170,t171,t172,t173,t174,t175,t176,t177,t178,t1782,t1784,t1786,t1788,t179,t18,t180,t181,t182,t183,t184,t185,t186,t187,t188,t189,t190,t191,t192,t193,t194,t195,t196,t1986,t1987,t2,t202,t203,t204,t205,t206,t208,t209,t211,t212,t213,t214,t215,t216,t218,t219,t220,t222,t223,t224,t226,t227,t230,t231,t233,t235,t236,t237,t238,t239,t241,t242,t243,t244,t245,t246,t247,t248,t253,t254,t255,t256,t257,t258,t259,t260,t261,t262,t265,t266,t268,t270,t272,t273,t274,t275,t276,t278,t280,t282,t283,t286,t291,t292,t293,t294,t295,t296,t297,t298,t3,t300,t301,t302,t304,t305,t306,t307,t308,t311,t313,t314,t315,t316,t317,t318,t319,t320,t323,t325,t326,t327,t328,t329,t33,t330,t331,t333,t334,t335,t337,t338,t339,t34,t340,t341,t342,t343,t344,t345,t346,t347,t348,t349,t35,t350,t351,t352,t353,t354,t355,t356,t357,t358,t359,t36,t360,t361,t362,t363,t364,t365,t366,t368,t369,t370,t372,t373,t374,t375,t376,t377,t378,t380,t381,t382,t383,t384,t385,t386,t387,t388,t389,t390,t391,t392,t393,t394,t395,t396,t397,t398,t399,t4,t40,t400,t401,t402,t403,t404,t405,t408,t409,t41,t410,t411,t412,t413,t414,t415,t417,t418,t419,t42,t420,t421,t422,t423,t425,t426,t427,t428,t429,t43,t430,t431,t432,t433,t434,t435,t44,t441,t442,t443,t444,t445,t447,t45,t454,t455,t456,t457,t459,t46,t460,t462,t463,t466,t467,t47,t471,t472,t473,t474,t475,t476,t477,t478,t479,t48,t480,t481,t482,t483,t484,t485,t486,t487,t488,t489,t49,t491,t493,t495,t496,t497,t498,t499,t5,t50,t501,t504,t505,t506,t507,t508,t509,t51,t510,t511,t512,t513,t52,t522,t523,t526,t527,t53,t530,t531,t535,t538,t539,t54,t540,t541,t545,t546,t547,t548,t549,t55,t551,t554,t557,t558,t559,t56,t560,t561,t562,t563,t565,t567,t57,t570,t571,t577,t58,t580,t586,t588,t59,t592,t593,t594,t595,t596,t597,t598,t599,t6,t60,t600,t601,t602,t603,t604,t605,t606,t607,t608,t609,t61,t611,t612,t613,t614,t616,t62,t620,t621,t622,t623,t624,t626,t627,t628,t629,t63,t630,t631,t632,t633,t634,t635,t636,t637,t638,t639,t64,t646,t647,t648,t65,t652,t658,t659,t66,t660,t662,t663,t666,t667,t668,t669,t67,t670,t672,t673,t675,t676,t677,t678,t68,t681,t682,t683,t684,t685,t686,t687,t688,t689,t69,t690,t697,t698,t699,t7,t70,t701,t702,t704,t705,t706,t71,t711,t712,t713,t715,t716,t718,t719,t72,t720,t727,t728,t729,t73,t730,t731,t735,t736,t737,t738,t739,t74,t742,t743,t747,t748,t764,t765,t766,t767,t773,t774,t778,t779,t780,t781,t782,t783,t784,t785,t787,t788,t790,t791,t792,t793,t794,t795,t797,t798,t799,t8,t800,t802,t803,t804,t805,t806,t808,t809,t81,t810,t811,t813,t814,t815,t816,t818,t819,t82,t820,t821,t822,t823,t824,t825,t826,t827,t828,t829,t83,t830,t832,t833,t834,t835,t836,t837,t838,t839,t84,t840,t841,t842,t843,t844,t845,t846,t847,t848,t849,t85,t850,t851,t852,t853,t854,t856,t858,t859,t86,t860,t862,t864,t867,t868,t87,t870,t872,t873,t874,t877,t878,t879,t88,t880,t882,t883,t884,t885,t887,t888,t889,t89,t890,t891,t892,t893,t895,t896,t897,t899,t9,t90,t900,t901,t902,t903,t904,t905,t906,t91,t911,t912,t913,t914,t915,t916,t917,t918,t919,t92,t920,t921,t922,t923,t924,t925,t926,t927,t928,t931,t932,t933,t935,t938,t939,t940,t942,t943,t944,t945,t947,t948,t949,t95,t951,t952,t953,t954,t955,t956,t957,t958,t959,t966,t967,t968,t969,t970,t971,t972,t973,t975,t976,t979,t981,t987,t988,t992,t993,t995,t996,t997,t998,t999] = ct{:};
t1127 = t5.*t513.*2.0;
t1130 = t3.*t10.*t11.*t115;
t1131 = t4.*t9.*t11.*t115;
t1138 = t3.*t5.*t10.*t11.*t51;
t1139 = t4.*t5.*t9.*t11.*t51;
t1140 = t3.*t5.*t10.*t12.*t51;
t1141 = t4.*t5.*t9.*t12.*t51;
t1144 = t3.*t5.*t10.*t11.*t52;
t1145 = t4.*t5.*t9.*t11.*t52;
t1146 = t3.*t5.*t10.*t11.*t53;
t1147 = t4.*t5.*t9.*t11.*t53;
t1163 = t5.*t698;
t1164 = t5.*t699;
t1168 = t3.*t4.*t316;
t1172 = t3.*t4.*t318;
t1174 = t5.*t712;
t1175 = t5.*t713;
t1179 = t3.*t4.*t328;
t1183 = t3.*t4.*t330;
t1185 = t5.*t728;
t1187 = t5.*t729;
t1199 = t5.*t736;
t1201 = t5.*t737;
t1215 = t35.*t36.*t51;
t1217 = t34.*t36.*t54;
t1222 = t3.*t10.*t11.*t135;
t1223 = t4.*t9.*t11.*t135;
t1235 = t3.*t10.*t11.*t141;
t1236 = t4.*t9.*t11.*t141;
t1254 = t9.*t10.*t333;
t1255 = t9.*t10.*t334;
t1256 = t9.*t10.*t337;
t1257 = t9.*t10.*t338;
t1259 = t36.*t218.*2.0;
t1260 = t36.*t222.*2.0;
t1261 = t34.*t237.*2.0;
t1262 = t34.*t238.*2.0;
t1264 = t36.*t242.*2.0;
t1265 = Lxcm6.*Lycm6.*m6.*t7.*t13.*t34.*2.0;
t1266 = Lxcm6.*Lycm6.*m6.*t7.*t13.*t35.*2.0;
t1267 = t35.*t254.*2.0;
t1268 = Lxcm5.*Lzcm5.*m5.*t6.*t12.*t34.*2.0;
t1269 = t35.*t258.*2.0;
t1273 = t3.*t4.*t36.*t54;
t1278 = t3.*t6.*t7.*t10.*t13.*t40;
t1279 = t4.*t6.*t7.*t9.*t13.*t40;
t1281 = t5.*t824;
t1282 = t5.*t825;
t1285 = t6.*t838;
t1287 = t3.*t10.*t11.*t206;
t1288 = t4.*t9.*t11.*t206;
t1289 = t5.*t9.*t10.*t206;
t1291 = t6.*t848;
t1292 = t6.*t849;
t1293 = t6.*t850;
t1294 = t6.*t851;
t1295 = t6.*t854;
t1298 = t6.*t856;
t1302 = t6.*t868;
t1305 = t6.*t870;
t1320 = t5.*t9.*t10.*t233;
t1321 = t6.*t900;
t1322 = t6.*t926;
t1324 = t6.*t927;
t1337 = t7.*t12.*t13.*t261;
t1338 = t7.*t12.*t13.*t262;
t1340 = t3.*t10.*t11.*t268;
t1341 = t4.*t9.*t11.*t268;
t1343 = t6.*t952;
t1345 = t3.*t10.*t12.*t280;
t1346 = t4.*t9.*t12.*t280;
t1355 = -t778;
t1356 = -t779;
t1366 = -t805;
t1367 = -t806;
t1369 = -t810;
t1370 = -t811;
t1377 = -t824;
t1378 = -t825;
t1382 = -t829;
t1383 = -t830;
t1386 = -t834;
t1388 = -t838;
t1389 = -t841;
t1391 = -t843;
t1395 = -t848;
t1396 = -t849;
t1397 = -t850;
t1398 = -t851;
t1420 = -t891;
t1421 = -t892;
t1422 = -t893;
t1424 = -t895;
t1425 = -t896;
t1426 = -t897;
t1428 = -t902;
t1432 = -t1132;
t1434 = -t914;
t1436 = -t918;
t1437 = -t919;
t1438 = -t920;
t1440 = -t925;
t1441 = -t926;
t1442 = -t927;
t1450 = -t1134;
t1461 = t3.*t4.*t383;
t1462 = t3.*t4.*t385;
t1463 = t3.*t4.*t387;
t1464 = t3.*t4.*t389;
t1465 = t3.*t4.*t393;
t1468 = -t1169;
t1469 = -t1170;
t1470 = t3.*t4.*t395;
t1471 = t3.*t4.*t399;
t1474 = -t1180;
t1475 = -t1181;
t1476 = t3.*t4.*t401;
t1477 = Lz5.*Lzcm6.*m6.*t34.*t35.*-2.0;
t1499 = Ixz6.*t3.*t5.*t7.*t10.*t35;
t1500 = Ixz6.*t4.*t5.*t7.*t9.*t35;
t1506 = Izx6.*t3.*t5.*t7.*t10.*t35;
t1507 = Izx6.*t4.*t5.*t7.*t9.*t35;
t1508 = t5.*t1095;
t1517 = t5.*t1098;
t1535 = Iyz6.*t3.*t5.*t10.*t13.*t35;
t1536 = Iyz6.*t3.*t7.*t10.*t12.*t34;
t1537 = Iyz6.*t4.*t5.*t9.*t13.*t35;
t1538 = Iyz6.*t4.*t7.*t9.*t12.*t34;
t1540 = Izy6.*t3.*t5.*t10.*t13.*t35;
t1541 = Izy6.*t3.*t7.*t10.*t12.*t34;
t1542 = Izy6.*t4.*t5.*t9.*t13.*t35;
t1543 = Izy6.*t4.*t7.*t9.*t12.*t34;
t1552 = Ixz6.*t3.*t10.*t12.*t13.*t34;
t1553 = Ixz6.*t4.*t9.*t12.*t13.*t34;
t1559 = Izx6.*t3.*t10.*t12.*t13.*t34;
t1560 = Izx6.*t4.*t9.*t12.*t13.*t34;
t1564 = Lz5.*Lzcm6.*m6.*t3.*t4.*t35.*-2.0;
t1579 = t3.*t4.*t5.*t206;
t1594 = t6.*t802;
t1595 = t6.*t803;
t1597 = t6.*t805;
t1598 = t6.*t806;
t1600 = t6.*t810;
t1601 = t6.*t811;
t1605 = t3.*t6.*t10.*t12.*t115;
t1606 = t4.*t6.*t9.*t12.*t115;
t1612 = t6.*t7.*t11.*t13.*t85.*2.0;
t1638 = t6.*t11.*t12.*t381;
t1649 = t6.*t1169;
t1650 = t6.*t1170;
t1652 = t6.*t1180;
t1653 = t6.*t1181;
t1690 = t149+t150;
t1691 = t153+t154;
t1697 = t34.*t472.*2.0;
t1698 = t34.*t473.*2.0;
t1699 = t34.*t475.*2.0;
t1700 = t34.*t476.*2.0;
t1702 = t36.*t475.*2.0;
t1703 = t36.*t476.*2.0;
t1704 = t5.*t36.*t242.*4.0;
t1707 = t35.*t498.*2.0;
t1708 = t35.*t499.*2.0;
t1711 = t34.*t546.*2.0;
t1712 = t34.*t547.*2.0;
t1716 = t3.*t10.*t11.*t36.*t51;
t1717 = t4.*t9.*t11.*t36.*t51;
t1732 = -t1286;
t1748 = t3.*t4.*t1023;
t1755 = -t1610;
t1756 = -t1611;
t1777 = -t1354;
t1783 = t3.*t10.*t11.*t385;
t1785 = t4.*t9.*t11.*t385;
t1787 = t3.*t10.*t11.*t389;
t1789 = t4.*t9.*t11.*t389;
t1791 = t3.*t10.*t11.*t395;
t1792 = t4.*t9.*t11.*t395;
t1793 = t3.*t10.*t11.*t401;
t1794 = t4.*t9.*t11.*t401;
t1823 = t6.*t34.*t282.*-2.0;
t1824 = t6.*t34.*t286.*-2.0;
t1828 = t6.*t11.*t12.*t454;
t1829 = t3.*t6.*t10.*t12.*t219;
t1830 = t4.*t6.*t9.*t12.*t219;
t1831 = t3.*t5.*t10.*t11.*t220;
t1832 = t4.*t5.*t9.*t11.*t220;
t1833 = t6.*t11.*t12.*t456;
t1834 = t3.*t6.*t10.*t12.*t223;
t1835 = t4.*t6.*t9.*t12.*t223;
t1836 = t3.*t5.*t10.*t11.*t224;
t1837 = t4.*t5.*t9.*t11.*t224;
t1840 = t3.*t5.*t10.*t11.*t270;
t1841 = t4.*t5.*t9.*t11.*t270;
t1842 = t3.*t5.*t10.*t11.*t272;
t1843 = t4.*t5.*t9.*t11.*t272;
t1845 = t6.*t11.*t12.*t551;
t1846 = t6.*t11.*t12.*t554;
t1879 = t35.*t805.*2.0;
t1880 = t35.*t806.*2.0;
t1882 = t35.*t810.*2.0;
t1883 = t35.*t811.*2.0;
t1886 = t34.*t824.*2.0;
t1887 = t34.*t825.*2.0;
t1889 = t35.*t854.*2.0;
t1891 = t35.*t856.*2.0;
t1894 = t35.*t868.*2.0;
t1896 = t35.*t870.*2.0;
t1904 = t35.*t1132;
t1935 = t3.*t5.*t6.*t10.*t12.*t95.*2.0;
t1936 = t4.*t5.*t6.*t9.*t12.*t95.*2.0;
t1953 = Lxcm6.*Lycm6.*m6.*t7.*t13.*t34.*t35.*-2.0;
t1958 = Lxcm6.*Lycm6.*m6.*t3.*t4.*t7.*t13.*t35.*-2.0;
t1970 = Lz5.*Lzcm6.*m6.*t3.*t5.*t10.*t11.*t35.*-2.0;
t1971 = Lz5.*Lzcm6.*m6.*t4.*t5.*t9.*t11.*t35.*-2.0;
t2026 = t34.*t36.*t475.*4.0;
t2027 = t34.*t36.*t476.*4.0;
t2067 = t35.*t1986;
t2068 = t35.*t1987;
t197 = -t101;
t198 = -t107;
t199 = -t108;
t200 = -t109;
t201 = -t110;
t406 = t3.*t4.*t108;
t407 = t3.*t4.*t110;
t416 = t5.*t190;
t424 = t5.*t192;
t438 = -t188;
t439 = -t191;
t440 = -t193;
t448 = t6.*t208;
t451 = t6.*t212;
t452 = -t194;
t453 = -t196;
t492 = t6.*t253;
t500 = t6.*t257;
t573 = -t359;
t574 = -t361;
t575 = -t362;
t576 = -t364;
t578 = t5.*t159;
t579 = t6.*t159;
t581 = t5.*t162;
t582 = t5.*t163;
t583 = t6.*t163;
t584 = t34.*t102;
t585 = t36.*t103;
t587 = t34.*t106;
t589 = t36.*t106;
t590 = t35.*t107;
t591 = t35.*t109;
t610 = t5.*t166;
t615 = t5.*t168;
t617 = t6.*t168;
t618 = t5.*t170;
t619 = t6.*t170;
t625 = -t273;
t640 = -t291;
t641 = -t293;
t642 = -t294;
t643 = -t296;
t644 = -t297;
t645 = -t298;
t649 = t36.*t121;
t650 = -t340;
t653 = -t346;
t654 = -t347;
t655 = -t348;
t656 = -t349;
t657 = -t350;
t664 = t3.*t4.*t120;
t665 = t3.*t4.*t122;
t674 = t9.*t10.*t120;
t679 = t9.*t10.*t122;
t680 = t11.*t12.*t122;
t693 = t6.*t301;
t696 = t6.*t305;
t709 = t6.*t315;
t723 = t6.*t327;
t751 = t9.*t10.*t190;
t752 = t9.*t10.*t191;
t753 = t9.*t10.*t192;
t754 = t9.*t10.*t193;
t755 = -t402;
t756 = -t404;
t757 = -t405;
t758 = -t417;
t759 = -t418;
t760 = -t421;
t761 = -t425;
t762 = -t426;
t763 = -t429;
t772 = -t647;
t775 = -t431;
t786 = t3.*t4.*t239;
t789 = t3.*t4.*t241;
t831 = t11.*t12.*t202;
t861 = t9.*t10.*t209;
t866 = t9.*t10.*t211;
t875 = t9.*t10.*t213;
t907 = t9.*t10.*t239;
t910 = t9.*t10.*t241;
t934 = t9.*t10.*t255;
t941 = t9.*t10.*t259;
t960 = t3.*t4.*t158;
t961 = -t447;
t963 = t3.*t4.*t161;
t964 = t3.*t4.*t162;
t974 = -t658;
t977 = t3.*t4.*t166;
t978 = -t659;
t980 = -t489;
t982 = -t491;
t984 = -t493;
t985 = -t662;
t986 = t3.*t4.*t169;
t990 = -t501;
t991 = -t663;
t994 = -t506;
t1006 = -t527;
t1016 = t11.*t12.*t159;
t1021 = -t667;
t1022 = t11.*t12.*t163;
t1030 = -t561;
t1034 = t11.*t12.*t168;
t1035 = -t571;
t1036 = t11.*t12.*t170;
t1077 = t3.*t4.*t190;
t1088 = t3.*t4.*t192;
t1115 = t9.*t10.*t344;
t1117 = t36.*t291;
t1118 = t9.*t10.*t350;
t1120 = t35.*t296;
t1121 = t35.*t297;
t1122 = t35.*t298;
t1128 = t11.*t12.*t208.*2.0;
t1129 = t11.*t12.*t212.*2.0;
t1133 = t11.*t12.*t253.*2.0;
t1135 = t11.*t12.*t257.*2.0;
t1142 = t5.*t676;
t1143 = t7.*t11.*t13.*t120;
t1148 = t3.*t10.*t12.*t121;
t1149 = t4.*t9.*t12.*t121;
t1150 = t7.*t12.*t13.*t121;
t1151 = t7.*t11.*t13.*t122;
t1152 = t3.*t10.*t11.*t123;
t1153 = t4.*t9.*t11.*t123;
t1154 = t3.*t10.*t11.*t124;
t1155 = t4.*t9.*t11.*t124;
t1156 = t3.*t10.*t11.*t125;
t1157 = t4.*t9.*t11.*t125;
t1162 = t3.*t4.*t311;
t1173 = t3.*t4.*t323;
t1189 = t9.*t10.*t300;
t1198 = t9.*t10.*t302;
t1203 = t9.*t10.*t304;
t1212 = t9.*t10.*t306;
t1213 = t34.*t346;
t1214 = t36.*t347;
t1216 = t34.*t350;
t1218 = t36.*t350;
t1219 = t35.*t351;
t1220 = t35.*t353;
t1221 = t35.*t355;
t1227 = t9.*t10.*t313;
t1233 = t9.*t10.*t317;
t1240 = t9.*t10.*t325;
t1246 = t9.*t10.*t329;
t1250 = -t681;
t1251 = -t684;
t1252 = -t689;
t1253 = -t690;
t1263 = t36.*t241.*2.0;
t1270 = t3.*t4.*t346;
t1271 = t36.*t373;
t1272 = t3.*t4.*t350;
t1274 = t3.*t4.*t352;
t1275 = t3.*t4.*t354;
t1276 = t3.*t4.*t356;
t1280 = t5.*t823;
t1290 = t3.*t4.*t540;
t1296 = t3.*t10.*t12.*t208;
t1299 = t4.*t9.*t12.*t208;
t1303 = t3.*t10.*t12.*t212;
t1306 = t4.*t9.*t12.*t212;
t1326 = t9.*t10.*t491;
t1327 = t3.*t10.*t12.*t253;
t1329 = t4.*t9.*t12.*t253;
t1332 = t3.*t10.*t12.*t257;
t1334 = t4.*t9.*t12.*t257;
t1339 = t9.*t10.*t506;
t1347 = t9.*t10.*t540;
t1348 = t3.*t4.*t577;
t1352 = t35.*t403;
t1353 = t36.*t404;
t1357 = -t782;
t1358 = -t783;
t1359 = -t784;
t1360 = -t785;
t1362 = -t790;
t1363 = -t791;
t1364 = t3.*t4.*t612;
t1365 = t3.*t4.*t613;
t1374 = -t814;
t1375 = t3.*t4.*t621;
t1376 = -t820;
t1379 = -t1127;
t1380 = -t826;
t1381 = -t827;
t1384 = -t832;
t1385 = -t833;
t1387 = -t837;
t1390 = -t842;
t1392 = -t845;
t1393 = -t846;
t1394 = -t847;
t1399 = t3.*t4.*t630;
t1400 = t3.*t10.*t11.*t159;
t1401 = t4.*t9.*t11.*t159;
t1402 = t3.*t4.*t631;
t1403 = t3.*t10.*t12.*t159;
t1404 = t4.*t9.*t12.*t159;
t1406 = t3.*t10.*t11.*t162;
t1407 = t4.*t9.*t11.*t162;
t1408 = t3.*t4.*t633;
t1409 = t3.*t10.*t11.*t163;
t1410 = t4.*t9.*t11.*t163;
t1411 = t3.*t4.*t634;
t1412 = t3.*t10.*t12.*t163;
t1413 = t4.*t9.*t12.*t163;
t1415 = t3.*t4.*t635;
t1416 = t3.*t4.*t636;
t1417 = t3.*t4.*t638;
t1418 = t35.*t431;
t1423 = t9.*t10.*t594;
t1427 = t9.*t10.*t597;
t1430 = t3.*t10.*t11.*t166;
t1431 = t4.*t9.*t11.*t166;
t1433 = -t913;
t1435 = -t917;
t1439 = -t924;
t1443 = t3.*t10.*t11.*t168;
t1444 = t4.*t9.*t11.*t168;
t1445 = -t931;
t1446 = t3.*t10.*t12.*t168;
t1447 = t4.*t9.*t12.*t168;
t1448 = -t935;
t1451 = t3.*t10.*t11.*t170;
t1452 = t4.*t9.*t11.*t170;
t1453 = -t938;
t1454 = t3.*t10.*t12.*t170;
t1455 = t4.*t9.*t12.*t170;
t1456 = -t942;
t1458 = t7.*t12.*t13.*t172;
t1459 = -t949;
t1495 = t5.*t1078;
t1496 = t5.*t1079;
t1497 = t3.*t4.*t419;
t1502 = t5.*t1089;
t1503 = t5.*t1090;
t1504 = t3.*t4.*t427;
t1526 = t3.*t5.*t10.*t11.*t102;
t1527 = t4.*t5.*t9.*t11.*t102;
t1530 = t3.*t5.*t10.*t11.*t106;
t1531 = t4.*t5.*t9.*t11.*t106;
t1532 = t3.*t10.*t11.*t189;
t1533 = t4.*t9.*t11.*t189;
t1534 = t3.*t4.*t434;
t1539 = t3.*t4.*t435;
t1544 = t3.*t5.*t10.*t11.*t108;
t1545 = t4.*t5.*t9.*t11.*t108;
t1546 = t3.*t5.*t10.*t11.*t110;
t1547 = t4.*t5.*t9.*t11.*t110;
t1548 = t3.*t10.*t11.*t190;
t1549 = t4.*t9.*t11.*t190;
t1551 = t9.*t10.*t419;
t1554 = t9.*t10.*t421;
t1555 = t3.*t10.*t11.*t192;
t1556 = t4.*t9.*t11.*t192;
t1558 = t9.*t10.*t427;
t1561 = t9.*t10.*t429;
t1562 = t9.*t10.*t434;
t1563 = t9.*t10.*t435;
t1567 = -t1075;
t1568 = -t1076;
t1569 = -t1078;
t1570 = -t1079;
t1571 = -t1259;
t1573 = -t1086;
t1574 = -t1087;
t1575 = -t1089;
t1576 = -t1090;
t1577 = -t1260;
t1582 = -t1264;
t1583 = -t1265;
t1584 = -t1267;
t1585 = -t1269;
t1586 = -t1101;
t1587 = -t1102;
out1 = ft_3({Ixx2,Ixx3,Ixx4,Ixx5,Ixx6,Ixy4,Ixy5,Ixy6,Ixz2,Ixz3,Ixz4,Ixz5,Ixz6,Iyx4,Iyx5,Iyx6,Iyy2,Iyy3,Iyy4,Iyy5,Iyy6,Iyz4,Iyz5,Iyz6,Izx2,Izx3,Izx4,Izx5,Izx6,Izy4,Izy5,Izy6,Izz1,Izz2,Izz3,Izz4,Izz5,Izz6,Lx3,Lxcm1,Lxcm2,Lxcm3,Lxcm4,Lxcm5,Lxcm6,Lycm1,Lycm2,Lycm3,Lycm4,Lycm5,Lycm6,Lz4,Lz5,Lzcm2,Lzcm3,Lzcm4,Lzcm5,Lzcm6,m1,m2,m3,m4,m5,m6,t10,t100,t1000,t1001,t1002,t1003,t1004,t1005,t1006,t1007,t1008,t1009,t1010,t1011,t1012,t1013,t1014,t1015,t1016,t1017,t1018,t1019,t102,t1020,t1021,t1022,t1023,t1024,t1025,t1026,t1027,t1028,t1029,t103,t1030,t1031,t1032,t1033,t1034,t1035,t1036,t1037,t1038,t1039,t104,t1040,t1041,t1042,t1047,t1048,t1049,t105,t1050,t1051,t1052,t1053,t1054,t1055,t1056,t1057,t1058,t1059,t106,t1060,t1061,t1062,t1063,t1064,t1065,t1066,t1067,t1068,t1069,t1070,t1071,t1072,t1073,t1074,t1075,t1076,t1077,t108,t1081,t1082,t1083,t1084,t1085,t1086,t1087,t1088,t1092,t1093,t1094,t1095,t1096,t1097,t1098,t1099,t11,t110,t1100,t1103,t1104,t1105,t1106,t1107,t1108,t1109,t111,t1110,t1111,t1112,t1113,t1114,t1115,t1117,t1118,t1119,t112,t1120,t1121,t1122,t1124,t1125,t1126,t1128,t1129,t113,t1130,t1131,t1133,t1135,t1136,t1137,t1138,t1139,t114,t1140,t1141,t1142,t1143,t1144,t1145,t1146,t1147,t1148,t1149,t115,t1150,t1151,t1152,t1153,t1154,t1155,t1156,t1157,t1162,t1163,t1164,t1168,t1172,t1173,t1174,t1175,t1179,t1183,t1185,t1187,t1189,t119,t1191,t1193,t1198,t1199,t12,t120,t1201,t1203,t1205,t1207,t121,t1212,t1213,t1214,t1215,t1216,t1217,t1218,t1219,t122,t1220,t1221,t1222,t1223,t1227,t123,t1233,t1235,t1236,t124,t1240,t1246,t125,t1250,t1251,t1252,t1253,t1254,t1255,t1256,t1257,t1261,t1262,t1263,t1266,t1268,t1270,t1271,t1272,t1273,t1274,t1275,t1276,t1278,t1279,t1280,t1281,t1282,t1285,t1287,t1288,t1289,t1290,t1291,t1292,t1293,t1294,t1295,t1296,t1298,t1299,t13,t1302,t1303,t1305,t1306,t1311,t1312,t1315,t1316,t1317,t1320,t1321,t1322,t1324,t1326,t1327,t1329,t1332,t1334,t1337,t1338,t1339,t134,t1340,t1341,t1343,t1344,t1345,t1346,t1347,t1348,t135,t1352,t1353,t1355,t1356,t1357,t1358,t1359,t1360,t1362,t1363,t1364,t1365,t1366,t1367,t1369,t1370,t1374,t1375,t1376,t1377,t1378,t1379,t138,t1380,t1381,t1382,t1383,t1384,t1385,t1386,t1387,t1388,t1389,t1390,t1391,t1392,t1393,t1394,t1395,t1396,t1397,t1398,t1399,t140,t1400,t1401,t1402,t1403,t1404,t1406,t1407,t1408,t1409,t141,t1410,t1411,t1412,t1413,t1415,t1416,t1417,t1418,t1420,t1421,t1422,t1423,t1424,t1425,t1426,t1427,t1428,t1430,t1431,t1432,t1433,t1434,t1435,t1436,t1437,t1438,t1439,t144,t1440,t1441,t1442,t1443,t1444,t1445,t1446,t1447,t1448,t1450,t1451,t1452,t1453,t1454,t1455,t1456,t1458,t1459,t146,t1461,t1462,t1463,t1464,t1465,t1466,t1467,t1468,t1469,t147,t1470,t1471,t1472,t1473,t1474,t1475,t1476,t1477,t1478,t1479,t148,t1480,t1481,t1482,t1483,t1484,t1485,t1486,t1487,t1488,t1489,t1490,t1491,t1492,t1493,t1495,t1496,t1497,t1499,t15,t1500,t1502,t1503,t1504,t1506,t1507,t1508,t1509,t151,t1510,t1511,t1512,t1513,t1514,t1515,t1516,t1517,t1518,t1519,t1520,t1521,t1522,t1523,t1524,t1525,t1526,t1527,t1530,t1531,t1532,t1533,t1534,t1535,t1536,t1537,t1538,t1539,t1540,t1541,t1542,t1543,t1544,t1545,t1546,t1547,t1548,t1549,t1551,t1552,t1553,t1554,t1555,t1556,t1558,t1559,t156,t1560,t1561,t1562,t1563,t1564,t1567,t1568,t1569,t157,t1570,t1571,t1573,t1574,t1575,t1576,t1577,t1579,t158,t1582,t1583,t1584,t1585,t1586,t1587,t159,t1594,t1595,t1597,t1598,t160,t1600,t1601,t1605,t1606,t161,t1612,t162,t163,t1638,t164,t1649,t165,t1650,t1652,t1653,t166,t167,t168,t169,t1690,t1691,t1697,t1698,t1699,t170,t1700,t1702,t1703,t1704,t1707,t1708,t171,t1711,t1712,t1716,t1717,t172,t173,t1732,t174,t1748,t175,t1755,t1756,t176,t177,t1777,t178,t1782,t1783,t1784,t1785,t1786,t1787,t1788,t1789,t179,t1791,t1792,t1793,t1794,t18,t180,t181,t182,t1823,t1824,t1828,t1829,t183,t1830,t1831,t1832,t1833,t1834,t1835,t1836,t1837,t184,t1840,t1841,t1842,t1843,t1845,t1846,t185,t186,t187,t1879,t188,t1880,t1882,t1883,t1886,t1887,t1889,t189,t1891,t1894,t1896,t190,t1904,t192,t1935,t1936,t195,t1953,t1958,t196,t197,t1970,t1971,t198,t1986,t1987,t199,t2,t200,t201,t202,t2026,t2027,t203,t204,t205,t206,t2067,t2068,t214,t215,t216,t218,t220,t222,t224,t226,t227,t230,t231,t235,t236,t239,t241,t242,t243,t244,t245,t246,t247,t248,t254,t256,t258,t260,t261,t262,t265,t266,t268,t270,t272,t274,t275,t276,t278,t280,t283,t292,t295,t296,t297,t298,t3,t301,t305,t307,t308,t311,t314,t315,t316,t318,t319,t320,t323,t326,t327,t328,t33,t330,t331,t335,t339,t34,t341,t342,t343,t344,t345,t346,t35,t350,t351,t352,t353,t354,t355,t356,t357,t358,t36,t360,t361,t363,t364,t365,t366,t368,t369,t370,t372,t373,t374,t375,t376,t377,t378,t380,t382,t383,t384,t385,t386,t387,t388,t389,t390,t391,t392,t393,t394,t395,t396,t397,t398,t399,t4,t40,t400,t401,t403,t405,t406,t407,t408,t409,t41,t410,t411,t412,t413,t414,t415,t416,t419,t42,t420,t422,t423,t424,t427,t428,t43,t430,t431,t432,t433,t434,t435,t438,t439,t44,t440,t441,t442,t443,t444,t445,t448,t45,t451,t452,t453,t454,t455,t456,t457,t459,t46,t460,t462,t463,t466,t467,t47,t471,t474,t475,t476,t477,t478,t479,t48,t480,t481,t482,t483,t484,t485,t486,t487,t488,t49,t492,t493,t495,t496,t497,t5,t50,t500,t501,t504,t505,t507,t508,t509,t51,t510,t511,t512,t52,t522,t523,t526,t53,t530,t531,t535,t538,t539,t54,t540,t541,t545,t548,t549,t55,t557,t558,t559,t56,t560,t562,t563,t565,t567,t57,t570,t571,t573,t574,t575,t576,t577,t578,t579,t58,t580,t581,t582,t583,t584,t585,t586,t587,t588,t589,t59,t590,t591,t592,t593,t594,t595,t596,t597,t598,t599,t6,t60,t600,t601,t602,t603,t604,t605,t606,t607,t608,t609,t61,t610,t611,t612,t613,t614,t615,t616,t617,t618,t619,t62,t620,t621,t622,t623,t624,t625,t626,t627,t628,t629,t63,t630,t631,t632,t633,t634,t635,t636,t637,t638,t639,t64,t640,t641,t642,t643,t644,t645,t646,t648,t649,t65,t650,t652,t653,t654,t655,t656,t657,t66,t660,t662,t663,t664,t665,t666,t668,t669,t67,t670,t672,t673,t674,t675,t676,t677,t678,t679,t68,t680,t681,t682,t683,t685,t686,t687,t688,t69,t693,t696,t697,t7,t70,t701,t702,t704,t705,t706,t709,t71,t711,t715,t716,t718,t719,t72,t720,t723,t727,t73,t730,t731,t735,t738,t739,t74,t742,t743,t747,t748,t751,t752,t753,t754,t755,t756,t757,t758,t759,t760,t761,t762,t763,t764,t765,t766,t767,t772,t773,t774,t775,t780,t781,t784,t786,t787,t788,t789,t790,t791,t792,t793,t794,t795,t797,t798,t799,t8,t800,t802,t803,t804,t808,t809,t81,t813,t815,t816,t818,t819,t82,t821,t822,t823,t828,t83,t831,t835,t836,t839,t84,t840,t844,t852,t853,t854,t856,t858,t859,t86,t860,t861,t862,t864,t866,t867,t868,t87,t870,t872,t873,t874,t875,t877,t878,t879,t88,t880,t882,t883,t884,t885,t887,t888,t889,t89,t890,t899,t9,t90,t900,t901,t903,t904,t905,t906,t907,t91,t910,t911,t912,t915,t916,t92,t921,t922,t923,t928,t931,t932,t933,t934,t935,t938,t939,t940,t941,t942,t943,t944,t945,t947,t948,t95,t951,t952,t953,t954,t955,t956,t957,t958,t959,t960,t961,t963,t964,t966,t967,t968,t969,t970,t971,t972,t973,t974,t975,t976,t977,t978,t979,t980,t981,t982,t984,t985,t986,t987,t988,t990,t991,t992,t993,t994,t995,t996,t997,t998,t999});
end
function out1 = ft_3(ct)
[Ixx2,Ixx3,Ixx4,Ixx5,Ixx6,Ixy4,Ixy5,Ixy6,Ixz2,Ixz3,Ixz4,Ixz5,Ixz6,Iyx4,Iyx5,Iyx6,Iyy2,Iyy3,Iyy4,Iyy5,Iyy6,Iyz4,Iyz5,Iyz6,Izx2,Izx3,Izx4,Izx5,Izx6,Izy4,Izy5,Izy6,Izz1,Izz2,Izz3,Izz4,Izz5,Izz6,Lx3,Lxcm1,Lxcm2,Lxcm3,Lxcm4,Lxcm5,Lxcm6,Lycm1,Lycm2,Lycm3,Lycm4,Lycm5,Lycm6,Lz4,Lz5,Lzcm2,Lzcm3,Lzcm4,Lzcm5,Lzcm6,m1,m2,m3,m4,m5,m6,t10,t100,t1000,t1001,t1002,t1003,t1004,t1005,t1006,t1007,t1008,t1009,t1010,t1011,t1012,t1013,t1014,t1015,t1016,t1017,t1018,t1019,t102,t1020,t1021,t1022,t1023,t1024,t1025,t1026,t1027,t1028,t1029,t103,t1030,t1031,t1032,t1033,t1034,t1035,t1036,t1037,t1038,t1039,t104,t1040,t1041,t1042,t1047,t1048,t1049,t105,t1050,t1051,t1052,t1053,t1054,t1055,t1056,t1057,t1058,t1059,t106,t1060,t1061,t1062,t1063,t1064,t1065,t1066,t1067,t1068,t1069,t1070,t1071,t1072,t1073,t1074,t1075,t1076,t1077,t108,t1081,t1082,t1083,t1084,t1085,t1086,t1087,t1088,t1092,t1093,t1094,t1095,t1096,t1097,t1098,t1099,t11,t110,t1100,t1103,t1104,t1105,t1106,t1107,t1108,t1109,t111,t1110,t1111,t1112,t1113,t1114,t1115,t1117,t1118,t1119,t112,t1120,t1121,t1122,t1124,t1125,t1126,t1128,t1129,t113,t1130,t1131,t1133,t1135,t1136,t1137,t1138,t1139,t114,t1140,t1141,t1142,t1143,t1144,t1145,t1146,t1147,t1148,t1149,t115,t1150,t1151,t1152,t1153,t1154,t1155,t1156,t1157,t1162,t1163,t1164,t1168,t1172,t1173,t1174,t1175,t1179,t1183,t1185,t1187,t1189,t119,t1191,t1193,t1198,t1199,t12,t120,t1201,t1203,t1205,t1207,t121,t1212,t1213,t1214,t1215,t1216,t1217,t1218,t1219,t122,t1220,t1221,t1222,t1223,t1227,t123,t1233,t1235,t1236,t124,t1240,t1246,t125,t1250,t1251,t1252,t1253,t1254,t1255,t1256,t1257,t1261,t1262,t1263,t1266,t1268,t1270,t1271,t1272,t1273,t1274,t1275,t1276,t1278,t1279,t1280,t1281,t1282,t1285,t1287,t1288,t1289,t1290,t1291,t1292,t1293,t1294,t1295,t1296,t1298,t1299,t13,t1302,t1303,t1305,t1306,t1311,t1312,t1315,t1316,t1317,t1320,t1321,t1322,t1324,t1326,t1327,t1329,t1332,t1334,t1337,t1338,t1339,t134,t1340,t1341,t1343,t1344,t1345,t1346,t1347,t1348,t135,t1352,t1353,t1355,t1356,t1357,t1358,t1359,t1360,t1362,t1363,t1364,t1365,t1366,t1367,t1369,t1370,t1374,t1375,t1376,t1377,t1378,t1379,t138,t1380,t1381,t1382,t1383,t1384,t1385,t1386,t1387,t1388,t1389,t1390,t1391,t1392,t1393,t1394,t1395,t1396,t1397,t1398,t1399,t140,t1400,t1401,t1402,t1403,t1404,t1406,t1407,t1408,t1409,t141,t1410,t1411,t1412,t1413,t1415,t1416,t1417,t1418,t1420,t1421,t1422,t1423,t1424,t1425,t1426,t1427,t1428,t1430,t1431,t1432,t1433,t1434,t1435,t1436,t1437,t1438,t1439,t144,t1440,t1441,t1442,t1443,t1444,t1445,t1446,t1447,t1448,t1450,t1451,t1452,t1453,t1454,t1455,t1456,t1458,t1459,t146,t1461,t1462,t1463,t1464,t1465,t1466,t1467,t1468,t1469,t147,t1470,t1471,t1472,t1473,t1474,t1475,t1476,t1477,t1478,t1479,t148,t1480,t1481,t1482,t1483,t1484,t1485,t1486,t1487,t1488,t1489,t1490,t1491,t1492,t1493,t1495,t1496,t1497,t1499,t15,t1500,t1502,t1503,t1504,t1506,t1507,t1508,t1509,t151,t1510,t1511,t1512,t1513,t1514,t1515,t1516,t1517,t1518,t1519,t1520,t1521,t1522,t1523,t1524,t1525,t1526,t1527,t1530,t1531,t1532,t1533,t1534,t1535,t1536,t1537,t1538,t1539,t1540,t1541,t1542,t1543,t1544,t1545,t1546,t1547,t1548,t1549,t1551,t1552,t1553,t1554,t1555,t1556,t1558,t1559,t156,t1560,t1561,t1562,t1563,t1564,t1567,t1568,t1569,t157,t1570,t1571,t1573,t1574,t1575,t1576,t1577,t1579,t158,t1582,t1583,t1584,t1585,t1586,t1587,t159,t1594,t1595,t1597,t1598,t160,t1600,t1601,t1605,t1606,t161,t1612,t162,t163,t1638,t164,t1649,t165,t1650,t1652,t1653,t166,t167,t168,t169,t1690,t1691,t1697,t1698,t1699,t170,t1700,t1702,t1703,t1704,t1707,t1708,t171,t1711,t1712,t1716,t1717,t172,t173,t1732,t174,t1748,t175,t1755,t1756,t176,t177,t1777,t178,t1782,t1783,t1784,t1785,t1786,t1787,t1788,t1789,t179,t1791,t1792,t1793,t1794,t18,t180,t181,t182,t1823,t1824,t1828,t1829,t183,t1830,t1831,t1832,t1833,t1834,t1835,t1836,t1837,t184,t1840,t1841,t1842,t1843,t1845,t1846,t185,t186,t187,t1879,t188,t1880,t1882,t1883,t1886,t1887,t1889,t189,t1891,t1894,t1896,t190,t1904,t192,t1935,t1936,t195,t1953,t1958,t196,t197,t1970,t1971,t198,t1986,t1987,t199,t2,t200,t201,t202,t2026,t2027,t203,t204,t205,t206,t2067,t2068,t214,t215,t216,t218,t220,t222,t224,t226,t227,t230,t231,t235,t236,t239,t241,t242,t243,t244,t245,t246,t247,t248,t254,t256,t258,t260,t261,t262,t265,t266,t268,t270,t272,t274,t275,t276,t278,t280,t283,t292,t295,t296,t297,t298,t3,t301,t305,t307,t308,t311,t314,t315,t316,t318,t319,t320,t323,t326,t327,t328,t33,t330,t331,t335,t339,t34,t341,t342,t343,t344,t345,t346,t35,t350,t351,t352,t353,t354,t355,t356,t357,t358,t36,t360,t361,t363,t364,t365,t366,t368,t369,t370,t372,t373,t374,t375,t376,t377,t378,t380,t382,t383,t384,t385,t386,t387,t388,t389,t390,t391,t392,t393,t394,t395,t396,t397,t398,t399,t4,t40,t400,t401,t403,t405,t406,t407,t408,t409,t41,t410,t411,t412,t413,t414,t415,t416,t419,t42,t420,t422,t423,t424,t427,t428,t43,t430,t431,t432,t433,t434,t435,t438,t439,t44,t440,t441,t442,t443,t444,t445,t448,t45,t451,t452,t453,t454,t455,t456,t457,t459,t46,t460,t462,t463,t466,t467,t47,t471,t474,t475,t476,t477,t478,t479,t48,t480,t481,t482,t483,t484,t485,t486,t487,t488,t49,t492,t493,t495,t496,t497,t5,t50,t500,t501,t504,t505,t507,t508,t509,t51,t510,t511,t512,t52,t522,t523,t526,t53,t530,t531,t535,t538,t539,t54,t540,t541,t545,t548,t549,t55,t557,t558,t559,t56,t560,t562,t563,t565,t567,t57,t570,t571,t573,t574,t575,t576,t577,t578,t579,t58,t580,t581,t582,t583,t584,t585,t586,t587,t588,t589,t59,t590,t591,t592,t593,t594,t595,t596,t597,t598,t599,t6,t60,t600,t601,t602,t603,t604,t605,t606,t607,t608,t609,t61,t610,t611,t612,t613,t614,t615,t616,t617,t618,t619,t62,t620,t621,t622,t623,t624,t625,t626,t627,t628,t629,t63,t630,t631,t632,t633,t634,t635,t636,t637,t638,t639,t64,t640,t641,t642,t643,t644,t645,t646,t648,t649,t65,t650,t652,t653,t654,t655,t656,t657,t66,t660,t662,t663,t664,t665,t666,t668,t669,t67,t670,t672,t673,t674,t675,t676,t677,t678,t679,t68,t680,t681,t682,t683,t685,t686,t687,t688,t69,t693,t696,t697,t7,t70,t701,t702,t704,t705,t706,t709,t71,t711,t715,t716,t718,t719,t72,t720,t723,t727,t73,t730,t731,t735,t738,t739,t74,t742,t743,t747,t748,t751,t752,t753,t754,t755,t756,t757,t758,t759,t760,t761,t762,t763,t764,t765,t766,t767,t772,t773,t774,t775,t780,t781,t784,t786,t787,t788,t789,t790,t791,t792,t793,t794,t795,t797,t798,t799,t8,t800,t802,t803,t804,t808,t809,t81,t813,t815,t816,t818,t819,t82,t821,t822,t823,t828,t83,t831,t835,t836,t839,t84,t840,t844,t852,t853,t854,t856,t858,t859,t86,t860,t861,t862,t864,t866,t867,t868,t87,t870,t872,t873,t874,t875,t877,t878,t879,t88,t880,t882,t883,t884,t885,t887,t888,t889,t89,t890,t899,t9,t90,t900,t901,t903,t904,t905,t906,t907,t91,t910,t911,t912,t915,t916,t92,t921,t922,t923,t928,t931,t932,t933,t934,t935,t938,t939,t940,t941,t942,t943,t944,t945,t947,t948,t95,t951,t952,t953,t954,t955,t956,t957,t958,t959,t960,t961,t963,t964,t966,t967,t968,t969,t970,t971,t972,t973,t974,t975,t976,t977,t978,t979,t980,t981,t982,t984,t985,t986,t987,t988,t990,t991,t992,t993,t994,t995,t996,t997,t998,t999] = ct{:};
t1588 = -t1103;
t1589 = -t1109;
t1590 = -t1112;
t1609 = -t1119;
t1615 = t3.*t4.*t675;
t1616 = t3.*t6.*t10.*t12.*t119;
t1617 = t4.*t6.*t9.*t12.*t119;
t1618 = t7.*t12.*t13.*t373;
t1619 = t3.*t7.*t10.*t13.*t120;
t1620 = t4.*t7.*t9.*t13.*t120;
t1625 = t3.*t7.*t10.*t13.*t122;
t1626 = t4.*t7.*t9.*t13.*t122;
t1627 = t6.*t11.*t12.*t376;
t1628 = t3.*t6.*t10.*t12.*t123;
t1629 = t4.*t6.*t9.*t12.*t123;
t1630 = t6.*t11.*t12.*t377;
t1631 = t3.*t6.*t10.*t12.*t124;
t1632 = t4.*t6.*t9.*t12.*t124;
t1633 = t6.*t11.*t12.*t378;
t1634 = t3.*t6.*t10.*t12.*t125;
t1635 = t4.*t6.*t9.*t12.*t125;
t1636 = t9.*t10.*t666;
t1637 = t9.*t10.*t668;
t1641 = t9.*t10.*t675;
t1644 = t9.*t10.*t681;
t1645 = t6.*t11.*t12.*t296;
t1646 = t6.*t11.*t12.*t297;
t1647 = t6.*t11.*t12.*t298;
t1655 = t3.*t10.*t12.*t301;
t1658 = t4.*t9.*t12.*t301;
t1662 = t3.*t10.*t12.*t305;
t1665 = t4.*t9.*t12.*t305;
t1668 = t3.*t10.*t12.*t315;
t1670 = t4.*t9.*t12.*t315;
t1673 = t3.*t10.*t12.*t327;
t1675 = t4.*t9.*t12.*t327;
t1678 = -t1138;
t1679 = -t1139;
t1680 = -t1140;
t1681 = -t1141;
t1683 = -t1144;
t1684 = -t1145;
t1685 = -t1146;
t1686 = -t1147;
t1692 = -t1215;
t1693 = -t1217;
t1701 = t36.*t474.*2.0;
t1705 = t34.*t662;
t1706 = t35.*t497.*2.0;
t1709 = t34.*t663;
t1714 = t36.*t562.*2.0;
t1715 = t35.*t571.*2.0;
t1718 = t11.*t12.*t36.*t120;
t1719 = t36.*t677;
t1720 = t36.*t678;
t1726 = t3.*t4.*t662;
t1727 = t3.*t4.*t663;
t1729 = -t1278;
t1730 = -t1279;
t1731 = -t1285;
t1733 = -t1289;
t1734 = -t1291;
t1735 = -t1292;
t1736 = -t1293;
t1737 = -t1294;
t1738 = -t1295;
t1740 = -t1298;
t1742 = t6.*t858.*-2.0;
t1743 = -t1302;
t1745 = -t1305;
t1747 = t6.*t872.*-2.0;
t1749 = t3.*t10.*t11.*t593;
t1750 = t4.*t9.*t11.*t593;
t1751 = t3.*t10.*t11.*t596;
t1752 = t4.*t9.*t11.*t596;
t1753 = t3.*t10.*t11.*t604;
t1754 = t4.*t9.*t11.*t604;
t1757 = -t1612;
t1758 = -t1322;
t1759 = t3.*t10.*t12.*t614;
t1760 = -t1324;
t1761 = t4.*t9.*t12.*t614;
t1764 = t6.*t935.*-2.0;
t1767 = t6.*t942.*-2.0;
t1769 = t6.*t7.*t11.*t13.*t121.*2.0;
t1770 = -t1337;
t1771 = -t1338;
t1774 = t3.*t4.*t1039;
t1775 = t3.*t4.*t1042;
t1778 = t3.*t4.*t1053;
t1779 = t3.*t4.*t1061;
t1790 = t35.*t36.*t172;
t1795 = t6.*t11.*t12.*t403;
t1796 = t3.*t6.*t10.*t12.*t188;
t1797 = t4.*t6.*t9.*t12.*t188;
t1798 = t6.*t11.*t12.*t405;
t1799 = t3.*t6.*t10.*t12.*t189;
t1800 = t4.*t6.*t9.*t12.*t189;
t1801 = t6.*t11.*t12.*t431;
t1807 = -t1699;
t1808 = -t1700;
t1809 = -t1702;
t1810 = -t1703;
t1811 = -t1704;
t1819 = -t1535;
t1820 = -t1537;
t1821 = -t1540;
t1822 = -t1542;
t1849 = t3.*t4.*t5.*t604;
t1850 = t6.*t1356;
t1868 = t148+t339;
t1875 = t36.*t790.*2.0;
t1876 = t36.*t791.*2.0;
t1878 = t35.*t804.*2.0;
t1881 = t35.*t809.*2.0;
t1884 = t3.*t6.*t7.*t10.*t13.*t103.*2.0;
t1885 = t4.*t6.*t7.*t9.*t13.*t103.*2.0;
t1888 = t35.*t853.*2.0;
t1890 = t34.*t859.*2.0;
t1892 = t34.*t860.*2.0;
t1893 = t35.*t867.*2.0;
t1895 = t34.*t873.*2.0;
t1897 = t34.*t874.*2.0;
t1900 = t147+t357;
t1901 = t3.*t10.*t11.*t646;
t1902 = t4.*t9.*t11.*t646;
t1905 = t34.*t932.*2.0;
t1906 = t34.*t933.*2.0;
t1907 = t35.*t931.*2.0;
t1908 = t34.*t939.*2.0;
t1909 = t34.*t940.*2.0;
t1910 = t35.*t938.*2.0;
t1911 = t3.*t10.*t11.*t35.*t119;
t1912 = t4.*t9.*t11.*t35.*t119;
t1913 = t3.*t10.*t11.*t648;
t1914 = t4.*t9.*t11.*t648;
t1915 = t3.*t10.*t11.*t35.*t121;
t1916 = t4.*t9.*t11.*t35.*t121;
t1925 = t35.*t953.*2.0;
t1926 = t35.*t955.*2.0;
t1927 = t151+t358;
t1941 = t3.*t6.*t7.*t10.*t13.*t121;
t1942 = t4.*t6.*t7.*t9.*t13.*t121;
t1943 = t3.*t7.*t10.*t13.*t292;
t1944 = t4.*t7.*t9.*t13.*t292;
t1946 = t3.*t7.*t10.*t13.*t295;
t1947 = t4.*t7.*t9.*t13.*t295;
t1949 = t36.*t1075.*2.0;
t1950 = t36.*t1076.*2.0;
t1951 = t36.*t1086.*2.0;
t1952 = t36.*t1087.*2.0;
t1966 = -t1889;
t1967 = -t1891;
t1968 = -t1894;
t1969 = -t1896;
t1973 = t6.*t11.*t12.*t36.*t172;
t1976 = t6.*t1690;
t1977 = t12.*t1690;
t1978 = t6.*t1691;
t1979 = t12.*t1691;
t1984 = -t1828;
t1985 = -t1833;
t1988 = -t1840;
t1989 = -t1841;
t1990 = -t1842;
t1991 = -t1843;
t1997 = t3.*t5.*t10.*t12.*t36.*t120;
t1998 = t4.*t5.*t9.*t12.*t36.*t120;
t2013 = t6.*t7.*t11.*t13.*t474.*2.0;
t2014 = t3.*t6.*t7.*t10.*t13.*t241.*2.0;
t2015 = t4.*t6.*t7.*t9.*t13.*t241.*2.0;
t2016 = t3.*t5.*t10.*t12.*t493.*2.0;
t2017 = t4.*t5.*t9.*t12.*t493.*2.0;
t2018 = t3.*t5.*t10.*t12.*t501.*2.0;
t2019 = t4.*t5.*t9.*t12.*t501.*2.0;
t2020 = t3.*t5.*t10.*t12.*t541.*2.0;
t2021 = t4.*t5.*t9.*t12.*t541.*2.0;
t2022 = t3.*t5.*t10.*t12.*t549.*2.0;
t2023 = t4.*t5.*t9.*t12.*t549.*2.0;
t2024 = t6.*t7.*t11.*t13.*t562.*2.0;
t2087 = t159+t163+t168+t170+t177+t181+t184+t187;
t2088 = t42+t120+t122+t256+t260+t318+t330+t410+t413+t631+t634;
t776 = t9.*t10.*t199;
t777 = t9.*t10.*t201;
t962 = t6.*t578;
t965 = t6.*t582;
t983 = t6.*t615;
t989 = t6.*t618;
t1043 = -t584;
t1044 = -t585;
t1045 = -t587;
t1046 = -t589;
t1123 = -t649;
t1248 = -t674;
t1249 = -t679;
t1283 = -t751;
t1284 = -t753;
t1301 = t9.*t10.*t448;
t1308 = t9.*t10.*t451;
t1331 = t9.*t10.*t492;
t1336 = t9.*t10.*t500;
t1349 = t3.*t4.*t579;
t1350 = t3.*t4.*t581;
t1351 = t3.*t4.*t583;
t1361 = t3.*t4.*t610;
t1368 = t3.*t4.*t617;
t1371 = t3.*t4.*t619;
t1405 = -t1128;
t1414 = -t1129;
t1429 = -t907;
t1449 = -t1133;
t1457 = -t1135;
t1460 = t11.*t12.*t625;
t1494 = t3.*t4.*t416;
t1501 = t3.*t4.*t424;
t1550 = t9.*t10.*t416;
t1557 = t9.*t10.*t424;
t1566 = t36.*t587;
t1572 = t3.*t4.*t439;
t1578 = t3.*t4.*t440;
t1607 = t9.*t10.*t653;
t1608 = t9.*t10.*t657;
t1621 = t11.*t12.*t665;
t1622 = t6.*t1148;
t1623 = t6.*t1149;
t1643 = t11.*t12.*t679;
t1660 = t9.*t10.*t693;
t1667 = t9.*t10.*t696;
t1672 = t9.*t10.*t709;
t1677 = t9.*t10.*t723;
t1682 = -t1143;
t1687 = -t1148;
t1688 = -t1149;
t1689 = -t1150;
t1694 = -t1219;
t1695 = -t1220;
t1696 = -t1221;
t1721 = t36.*t680;
t1722 = -t1271;
t1723 = -t1274;
t1724 = -t1275;
t1725 = -t1276;
t1728 = t3.*t4.*t994;
t1739 = t3.*t10.*t11.*t579;
t1741 = t4.*t9.*t11.*t579;
t1744 = t3.*t10.*t11.*t583;
t1746 = t4.*t9.*t11.*t583;
t1762 = t3.*t10.*t11.*t617;
t1763 = t4.*t9.*t11.*t617;
t1765 = t3.*t10.*t11.*t619;
t1766 = t4.*t9.*t11.*t619;
t1768 = t5.*t1143.*2.0;
t1772 = t5.*t1458;
t1773 = -t1347;
t1776 = -t1352;
t1780 = t35.*t759;
t1781 = t35.*t762;
t1803 = -t1497;
t1804 = t3.*t4.*t760;
t1805 = -t1504;
t1806 = t3.*t4.*t763;
t1812 = -t1706;
t1813 = -t1526;
t1814 = -t1527;
t1815 = t3.*t10.*t11.*t438;
t1816 = t4.*t9.*t11.*t438;
t1817 = -t1530;
t1818 = -t1531;
t1827 = -t1714;
t1838 = -t1562;
t1839 = -t1563;
t1851 = t3.*t4.*t982;
t1855 = t35.*t1271;
t1857 = -t1616;
t1858 = -t1617;
t1859 = -t1619;
t1860 = -t1620;
t1864 = t3.*t4.*t1250;
t1865 = -t1627;
t1866 = -t1630;
t1867 = -t1633;
t1870 = t36.*t1118;
t1871 = -t1641;
t1872 = t7.*t12.*t13.*t640;
t1874 = t36.*t789.*2.0;
t1903 = t36.*t910.*2.0;
t1919 = t35.*t1152;
t1920 = t35.*t1153;
t1921 = t35.*t1154;
t1922 = t35.*t1155;
t1923 = t35.*t1156;
t1924 = t35.*t1157;
t1928 = t35.*t1214;
t1930 = -t1719;
t1931 = -t1720;
t1937 = t5.*t1618;
t1938 = t5.*t1619;
t1939 = t5.*t1620;
t1948 = t9.*t10.*t1150;
t1959 = -t1878;
t1960 = -t1881;
t1961 = -t1795;
t1962 = -t1884;
t1963 = -t1885;
t1964 = -t1799;
t1965 = -t1800;
t1974 = -t1925;
t1975 = -t1926;
t1982 = t3.*t5.*t10.*t11.*t589;
t1983 = t4.*t5.*t9.*t11.*t589;
t1992 = t3.*t4.*t36.*t657;
t1993 = Lx3.*t1900;
t1994 = t146+t650;
t1995 = t35.*t36.*t640;
t1996 = t11.*t12.*t36.*t664;
t2000 = t3.*t6.*t10.*t12.*t649;
t2001 = t4.*t6.*t9.*t12.*t649;
t2002 = Lx3.*t1927;
t2025 = t34.*t36.*t657;
t2029 = -t1941;
t2030 = -t1942;
t2032 = -t1946;
t2033 = -t1947;
t2034 = t35.*t1749;
t2035 = t35.*t1750;
t2036 = t35.*t1751;
t2037 = t35.*t1752;
t2038 = t34.*t1619.*2.0;
t2039 = t34.*t1620.*2.0;
t2040 = t34.*t1625.*2.0;
t2041 = t34.*t1626.*2.0;
t2042 = t7.*t1868;
t2043 = t13.*t1868;
t2044 = -t2013;
t2045 = t5.*t1900;
t2046 = -t2020;
t2047 = -t2021;
t2048 = -t2022;
t2049 = -t2023;
t2050 = t11.*t1900;
t2051 = t5.*t1927;
t2052 = t11.*t1927;
t2055 = -t1997;
t2056 = -t1998;
t2061 = t35.*t1913;
t2062 = t35.*t1914;
t2089 = t84+t135+t141+t162+t166+t176+t180+t182+t185+t190+t192+t268+t385+t389+t395+t401+t579+t583+t617+t619+t621+t646+t676+t1250;
t2090 = t100+t280+t292+t295+t384+t388+t394+t400+t541+t549+t578+t582+t606+t614+t615+t618+t629+t731+t739+t961+t980+t984+t990+t1054+t1062;
t1825 = -t1550;
t1826 = -t1557;
t1844 = t35.*t1044;
t1847 = t3.*t4.*t962;
t1848 = t3.*t4.*t965;
t1852 = t3.*t4.*t983;
t1853 = t3.*t4.*t989;
t1861 = -t1768;
t1862 = -t1622;
t1863 = -t1623;
t1873 = t11.*t12.*t1249;
t1932 = -t1721;
t1972 = -t1903;
t1999 = t36.*t1621;
t2004 = t36.*t1643;
t2005 = t3.*t10.*t11.*t1123;
t2006 = t4.*t9.*t11.*t1123;
t2007 = -t1919;
t2008 = -t1920;
t2009 = -t1921;
t2010 = -t1922;
t2011 = -t1923;
t2012 = -t1924;
t2028 = t3.*t4.*t1689;
t2031 = t5.*t1872;
t2053 = t35.*t1815;
t2054 = t35.*t1816;
t2058 = -t2040;
t2059 = -t2041;
t2060 = t11.*t12.*t36.*t1248;
t2071 = t64+t2050;
t2072 = t63+t2051;
t2077 = t341+t2043;
t2079 = -t12.*(t65-t2045);
t2082 = t6.*(t65-t2045);
t2091 = t559+t973+t1011+t1012+t1360+t1392+t2090;
t2092 = t40+t41+t74+t88+t91+t92+t115+t119+t121+t123+t124+t125+t189+t206+t214+t215+t216+t242+t314+t326+t392+t398+t408+t411+t438+t507+t539+t593+t596+t604+t609+t611+t632+t648+t758+t761+t979+t981+t995+t1016+t1022+t1034+t1036+t1067+t1072+t1097+t1100+t1123+t1151+t1582+t1682;
t2096 = t202+t444+t625+t664+t665+t765+t802+t803+t808+t813+t899+t954+t956+t968+t1002+t1003+t1172+t1183+t1248+t1249+t1255+t1257+t1321+t1343+t1355+t1358+t1389+t1390+t1395+t1397+t1400+t1401+t1402+t1409+t1410+t1411+t1443+t1444+t1448+t1451+t1452+t1456+t1481+t1482+t1483+t1489+t1490+t1491+t1511+t1512+t1516+t1520+t1521+t1525+t1597+t1598+t1600+t1601+t1649+t1650+t1652+t1653+t1680+t1681+t1687+t1688+t1731+t1735+t1737+t1738+t1740+t1743+t1745+t1758+t1760+t1782+t1784+t1786+t1788+t1850;
t2098 = t261+t262+t265+t266+t471+t478+t482+t486+t548+t562+t669+t670+t672+t673+t677+t678+t682+t683+t685+t686+t687+t688+t697+t711+t730+t738+t742+t747+t787+t788+t793+t795+t800+t823+t861+t862+t864+t875+t878+t880+t883+t885+t888+t890+t901+t934+t941+t944+t951+t964+t977+t1005+t1030+t1038+t1041+t1049+t1057+t1077+t1088+t1095+t1098+t1104+t1105+t1163+t1164+t1174+t1175+t1185+t1187+t1198+t1199+t1201+t1212+t1233+t1246+t1281+t1282+t1283+t1284+t1296+t1299+t1303+t1306+t1317+t1327+t1329+t1332+t1334+t1344+t1345+t1346+t1349+t1351+t1362+t1363+t1368+t1371+t1375+t1386+t1391+t1420+t1421+t1424+t1425+t1434+t1436+t1437+t1438+t1440+t1458+t1462+t1464+t1466+t1467+t1470+t1472+t1473+t1476+t1495+t1496+t1502+t1503+t1586+t1587+t1618+t1644+t1655+t1658+t1662+t1665+t1668+t1670+t1673+t1675+t1701+t1716+t1717+t1729+t1730+t1732+t1755+t1756+t1759+t1761+t1777+t1827+t1864+t1872+t1875+t1876+t1930+t1931+t1938+t1939+t2029+t2030;
t2057 = -t1999;
t2069 = t35.*t2005;
t2070 = t35.*t2006;
t2075 = t12.*t2072;
t2076 = t6.*t2072;
t2085 = t1976+t2079;
t2086 = t1977+t2082;
t2093 = t205+t243+t245+t247+t445+t480+t484+t488+t903+t972+t1006+t1393+t2092;
t2094 = t95+t138+t144+t158+t161+t169+t175+t179+t183+t186+t239+t254+t258+t274+t275+t311+t316+t323+t328+t383+t387+t393+t399+t409+t412+t416+t424+t434+t435+t439+t440+t512+t540+t577+t581+t610+t612+t613+t620+t622+t630+t633+t635+t636+t638+t675+t680+t760+t763+t772+t962+t965+t982+t983+t989+t994+t1023+t1039+t1042+t1053+t1061+t1106+t1113+t1114+t1142+t1251+t1252+t1253+t1263+t1422+t1426+t1584+t1585+t1588+t1689+t1718+t1757+t1932;
t2097 = Ixx4+Iyy3+Izz5+Izz6+t46+t47+t48+t49+t50+t51+t52+t53+t54+t55+t56+t58+t59+t70+t71+t72+t73+t86+t87+t89+t90+t102+t103+t104+t105+t106+t111+t112+t113+t114+t164+t165+t167+t197+t198+t199+t200+t201+t204+t218+t222+t244+t246+t248+t270+t272+t343+t344+t345+t351+t352+t353+t354+t355+t356+t365+t368+t369+t370+t380+t419+t420+t427+t428+t443+t452+t453+t479+t483+t487+t560+t573+t574+t575+t576+t586+t588+t590+t591+t592+t594+t595+t597+t599+t602+t605+t616+t623+t624+t627+t628+t652+t653+t654+t655+t656+t657+t660+t666+t668+t759+t762+t767+t970+t974+t978+t985+t991+t996+t997+t1009+t1013+t1021+t1026+t1029+t1043+t1044+t1045+t1046+t1083+t1094+t1126+t1213+t1214+t1216+t1218+t1266+t1268+t1359+t1379+t1405+t1414+t1449+t1457+t1477+t1566+t1571+t1577+t1583+t1589+t1590+t1692+t1693+t1694+t1695+t1696+t1705+t1709+t1769+t1780+t1781+t1811+t1823+t1824+t1844+t1861+t1928+t1953+t2025;
et1 = t66+t67+t68+t171+t172+t173+t203+t366+t372+t373+t374+t375+t376+t377+t378+t403+t406+t407+t430+t432+t433+t441+t442+t454+t455+t456+t457+t477+t481+t485+t495+t496+t557+t558+t598+t601+t637+t639+t640+t641+t642+t643+t644+t645+t704+t705+t718+t719+t755+t756+t757+t764+t766+t773+t774+t775+t776+t777+t792+t794+t797+t798+t799+t815+t816+t821+t822+t854+t856+t868+t870+t877+t879+t882+t884+t887+t889+t900+t905+t906+t947+t948+t952+t966+t967+t969+t987+t988+t1004+t1008+t1014+t1015+t1017+t1018+t1024+t1025+t1027+t1028+t1051+t1052+t1059+t1060+t1063+t1064+t1068+t1069+t1081+t1082+t1092+t1093+t1115+t1117+t1120+t1121+t1122+t1124+t1125+t1191+t1193+t1205+t1207+t1222+t1223+t1235+t1236+t1270+t1272+t1273+t1320+t1340+t1341+t1353+t1356+t1357+t1366+t1367+t1369+t1370+t1380+t1381+t1382+t1383+t1384+t1385+t1387+t1388+t1396+t1398+t1406+t1407+t1418+t1423+t1427+t1430+t1431+t1432+t1433+t1435+t1439+t1441+t1442+t1450+t1468+t1469+t1474+t1475+t1478+t1479+t1486+t1487+t1499+t1500+t1506+t1507+t1509+t1510+t1518+t1519+t1548+t1549+t1551+t1555+t1556+t1558+t1564+t1579+t1594+t1595+t1605+t1606+t1607+t1608+t1609+t1628+t1629+t1631+t1632+t1634+t1635+t1636;
et2 = t1637+t1707+t1708+t1722+t1723+t1724+t1725+t1726+t1727+t1733+t1734+t1736+t1739+t1741+t1742+t1744+t1746+t1747+t1762+t1763+t1764+t1765+t1766+t1767+t1770+t1771+t1776+t1783+t1785+t1787+t1789+t1790+t1791+t1792+t1793+t1794+t1796+t1797+t1803+t1805+t1819+t1820+t1821+t1822+t1829+t1830+t1834+t1835+t1849+t1855+t1857+t1858+t1862+t1863+t1870+t1879+t1880+t1882+t1883+t1901+t1902+t1904+t1943+t1944+t1958+t1964+t1965+t1966+t1967+t1968+t1969+t1992+t1995+t2000+t2001+t2014+t2015+t2032+t2033+t2055+t2056;
t2099 = et1+et2;
t2080 = -t2076;
t2083 = t1978+t2075;
t2095 = t600+t603+t626+t904+t971+t1007+t1010+t1031+t1032+t1033+t1394+t2094;
et3 = t235+t236+t283+t307+t308+t319+t320+t331+t335+t382+t386+t390+t391+t396+t397+t414+t415+t422+t423+t459+t460+t462+t463+t475+t476+t497+t504+t505+t508+t509+t510+t511+t522+t523+t538+t545+t570+t580+t607+t608+t701+t702+t706+t715+t716+t720+t727+t735+t743+t748+t752+t754+t780+t781+t786+t804+t809+t818+t819+t828+t831+t835+t836+t839+t840+t852+t866+t910+t911+t912+t915+t916+t921+t922+t923+t928+t943+t945+t953+t955+t957+t958+t959+t960+t963+t975+t976+t986+t992+t993+t998+t999+t1000+t1001+t1019+t1020+t1035+t1037+t1040+t1047+t1048+t1050+t1055+t1056+t1058+t1065+t1066+t1070+t1071+t1073+t1074+t1084+t1085+t1096+t1099+t1107+t1108+t1110+t1111+t1130+t1131+t1136+t1137+t1152+t1153+t1154+t1155+t1156+t1157+t1162+t1168+t1173+t1179+t1189+t1203+t1227+t1240+t1254+t1256+t1261+t1262+t1280+t1287+t1288+t1290+t1301+t1308+t1311+t1312+t1315+t1316+t1326+t1331+t1336+t1339+t1348+t1350+t1361+t1364+t1365+t1374+t1376+t1377+t1378+t1399+t1403+t1404+t1408+t1412+t1413+t1415+t1416+t1417+t1429+t1445+t1446+t1447+t1453+t1454+t1455+t1459+t1460+t1461+t1463+t1465+t1471+t1480+t1484+t1485+t1488+t1492+t1493+t1494+t1501+t1508+t1513+t1514+t1515+t1517+t1522;
et4 = t1523+t1524+t1532+t1533+t1534+t1536+t1538+t1539+t1541+t1543+t1544+t1545+t1546+t1547+t1552+t1553+t1554+t1559+t1560+t1561+t1567+t1568+t1569+t1570+t1572+t1573+t1574+t1575+t1576+t1578+t1615+t1621+t1625+t1626+t1638+t1645+t1646+t1647+t1660+t1667+t1672+t1677+t1678+t1679+t1683+t1684+t1685+t1686+t1697+t1698+t1711+t1712+t1715+t1728+t1748+t1749+t1750+t1751+t1752+t1753+t1754+t1772+t1773+t1774+t1775+t1778+t1779+t1798+t1801+t1804+t1806+t1807+t1808+t1809+t1810+t1812+t1813+t1814+t1815+t1816+t1817+t1818+t1825+t1826+t1831+t1832+t1836+t1837+t1838+t1839+t1845+t1846+t1847+t1848+t1851+t1852+t1853+t1859+t1860+t1865+t1866+t1867+t1871+t1873+t1874+t1886+t1887+t1888+t1890+t1892+t1893+t1895+t1897+t1905+t1906+t1907+t1908+t1909+t1910+t1911+t1912+t1913+t1914+t1915+t1916+t1935+t1936+t1937+t1948+t1949+t1950+t1951+t1952+t1959+t1960+t1961+t1962+t1963+t1970+t1971+t1972+t1973+t1974+t1975+t1982+t1983+t1984+t1985+t1986+t1987+t1988+t1989+t1990+t1991+t1996+t2004+t2005+t2006+t2007+t2008+t2009+t2010+t2011+t2012+t2016+t2017+t2018+t2019+t2024+t2026+t2027+t2028+t2031+t2034+t2035+t2036+t2037+t2038+t2039+t2044+t2046+t2047+t2048+t2049+t2053+t2054+t2057+t2058+t2059+t2060+t2061+t2062+t2067+t2068+t2069+t2070;
t2100 = et3+et4;
t2084 = t1979+t2080;
t2101 = t82+t83+t134+t140+t160+t174+t178+t226+t230+t276+t466+t526+t530+t563+t565+t567+t844+t1428+t2100;
et5 = Izz1+m6.*(t69+t1993+Lz4.*t1690+Lz5.*t2085+Lzcm6.*t2085-Lxcm6.*(t13.*t2071+t7.*t2086)-Lycm6.*(t7.*t2071-t13.*t2086)).^2+m3.*(t69-Lycm3.*t8+Lxcm3.*t2.*t43+Lzcm3.*t2.*t44).^2+m3.*(t81+Lycm3.*t2+Lxcm3.*t8.*t43+Lzcm3.*t8.*t44).^2+t9.*(Ixx2.*t9+Izx2.*t3)+t44.*(Ixx3.*t44+Izx3.*t43)+t3.*(Ixz2.*t9+Izz2.*t3)+t43.*(Ixz3.*t44+Izz3.*t43)+m6.*(t81+t2002+Lz4.*t1691+Lz5.*t2083+Lzcm6.*t2083-Lxcm6.*(t7.*t2084-t13.*(t62-t2052))+Lycm6.*(t13.*t2084+t7.*(t62-t2052))).^2+t43.*(Izz4.*t43+Ixz4.*t5.*t44-Iyz4.*t11.*t44);
et6 = m4.*(t69+t1993-Lycm4.*t2071-Lxcm4.*(t65-t2045)+Lzcm4.*t2.*t44).^2+m4.*(t81+t2002+Lxcm4.*t2072+Lycm4.*(t62-t2052)+Lzcm4.*t8.*t44).^2+m5.*(t81+Lycm5.*t62+Lx3.*t8.*t43+Lxcm5.*t6.*t63+Lz4.*t8.*t44+Lzcm5.*t12.*t63-Lxcm5.*t8.*t12.*t44+Lycm5.*t9.*t10.*t65+Lycm5.*t3.*t4.*t157+Lzcm5.*t6.*t8.*t44+Lxcm5.*t3.*t4.*t6.*t64-Lxcm5.*t6.*t9.*t10.*t64+Lzcm5.*t3.*t4.*t12.*t64-Lzcm5.*t9.*t10.*t12.*t64).^2+m5.*(t69-Lycm5.*t64+Lx3.*t2.*t43+Lxcm5.*t6.*t157+Lz4.*t2.*t44+Lzcm5.*t12.*t157-Lxcm5.*t2.*t12.*t44-Lycm5.*t3.*t4.*t63+Lycm5.*t9.*t10.*t63+Lzcm5.*t2.*t6.*t44+Lxcm5.*t3.*t4.*t6.*t62+Lxcm5.*t6.*t9.*t10.*t156+Lzcm5.*t3.*t4.*t12.*t62+Lzcm5.*t9.*t10.*t12.*t156).^2;
et7 = -t2077.*(-Iyy6.*t2077+Izy6.*t1994+Ixy6.*(t342-t2042))-t1994.*(Iyz6.*t2077-Izz6.*t1994+Ixz6.*(t342-t2042))+m1.*(Lxcm1.*t8+Lycm1.*t2).^2+m1.*(Lxcm1.*t2-Lycm1.*t8).^2+m2.*(-Lycm2.*t8+Lxcm2.*t2.*t3+Lzcm2.*t2.*t9).^2+m2.*(Lycm2.*t2+Lxcm2.*t3.*t8+Lzcm2.*t8.*t9).^2-(t342-t2042).*(Iyx6.*t2077+Izx6.*t1994-Ixx6.*(t342-t2042))+t1868.*(Ixx5.*t1868+Izx5.*t1994+Iyx5.*t11.*t44)+t1994.*(Ixz5.*t1868+Izz5.*t1994-Iyz5.*t11.*t44)+t11.*t44.*(Ixy5.*t1868-Izy5.*t1994+Iyy5.*t11.*t44)+t5.*t44.*(Izx4.*t43+Ixx4.*t5.*t44+Iyx4.*t11.*t44);
et8 = t11.*t44.*(-Izy4.*t43+Ixy4.*t5.*t44+Iyy4.*t11.*t44);
et9 = Ixx4+Iyy2+Iyy3+Izz5+Izz6+t46+t47+t48+t49+t50+t51+t52+t53+t54+t55+t56+t58+t59+t70.*2.0+t71.*2.0+t72.*2.0+t73.*2.0+t86.*2.0+t87.*2.0+t89.*2.0+t90.*2.0+t102+t103+t104+t105+t106+t111+t112+t113+t114+t164+t165+t167+t197+t198+t199+t200+t201+t204.*2.0+t218+t222-t227.*2.0-t231.*2.0+t244.*2.0+t246.*2.0+t248.*2.0+t270+t272-t278.*2.0+t343+t344+t345+t351+t352+t353+t354+t355+t356+t365+t368+t369+t370+t380+t419+t420+t427+t428+t443.*2.0+t452+t453-t467.*2.0+t479.*2.0+t483.*2.0+t487.*2.0-t531.*2.0-t535.*2.0+t560.*2.0+t573+t574+t575+t576+t586+t588+t590+t591+t592+t594+t595+t597+t605+t616+t623+t624+t628+t652+t653+t654+t655+t656+t657+t660+t666+t668+t759+t762+t767.*2.0-t784.*2.0+t974+t978+t985+t991+t996+t997+t1021+t1026+t1029+t1043+t1044+t1045+t1046+t1083+t1094+t1126+t1213+t1214+t1216+t1218+t1266+t1268+t1379+t1405+t1414+t1449+t1457+t1477+t1566+t1571+t1577;
et10 = t1583+t1589+t1590+t1692+t1693+t1694+t1695+t1696+t1705+t1709+t1769+t1780+t1781+t1811+t1823+t1824+t1844+t1861+t1928+t1953+t2025+m3.*t15+m4.*t15+m5.*t15+m6.*t15+Lxcm2.^2.*m2+Lzcm2.^2.*m2;
mt1 = [et5+et6+et7+et8,t2101,t2100,t2099,t2098,t2096,t2101,et9+et10,t2097,t2095,t2093,t2091,t2100,t2097,Ixx4+Iyy3+Izz5+Izz6+t46+t47+t48+t49+t50+t51+t52+t53+t54+t55+t56+t58+t59+t102+t103+t104+t105+t106+t111+t112+t113+t114+t164+t165+t167+t197+t198+t199+t200+t201+t218+t222+t270+t272+t343+t344+t345+t351+t352+t353+t354+t355+t356+t365+t368+t369+t370+t380+t419+t420+t427+t428+t452+t453+t573+t574+t575+t576+t586+t588+t590+t591+t592+t594+t595+t597+t605+t616+t623+t624+t628+t652+t653+t654+t655+t656+t657+t660+t666+t668+t759+t762+t974+t978+t985+t991+t996+t997+t1021+t1026+t1029+t1043+t1044+t1045+t1046+t1083+t1094+t1126+t1213+t1214+t1216+t1218+t1266+t1268+t1379+t1405+t1414+t1449+t1457+t1477+t1566+t1571+t1577+t1583+t1589+t1590+t1692+t1693+t1694+t1695+t1696+t1705+t1709+t1769+t1780+t1781+t1811+t1823+t1824+t1844+t1861+t1928+t1953+t2025,t2094,t2092,t2090,t2099,t2095,t2094];
mt2 = [Ixx5+Iyy6+Izz4+t45+t51+t52+t53+t57+t60+t61-t102-t106+t108+t110+t195+t196+t220+t224-t270-t272+t346+t350-t352-t354-t356+t360+t361+t363+t364-t419-t427-t586+t589+t662+t663-t666-t668+t1215-t1266+Ixx6.*t36-Iyy6.*t36+m4.*t18-t36.*t51+t36.*t54+t36.*t657-Lz5.*Lzcm6.*m6.*t35.*2.0,t2089,t2088,t2098,t2093,t2092,t2089,Ixx6./2.0+Iyy5+Iyy6./2.0+t45+t50+t51./2.0+t54./2.0+t57+t60+t61-t195-t360-t363-(Ixx6.*t33)./2.0+(Iyy6.*t33)./2.0+(t33.*t51)./2.0-(t33.*t54)./2.0,t2087,t2096,t2091,t2090,t2088,t2087,Izz6+t51+t54];
out1 = reshape([mt1,mt2],6,6);
end
